simulink model "active_vehicle_ESP_Control"  (R2020a)
settings: Solver=ode4  StartTime=0.0  StopTime=inf  FixedStep=1e-3  RelTol=1e-3
InitFcn:
  | clear mex
model workspace (MAT data in the model file):
  inChnlList{1} = 'Driver_Demands.str_swa'
  inChnlList{2} = 'Subsystem_Activation.Internal_Steering_Column_Activity'
  inChnlList{3} = 'Driver_Demands.rack_displacement'
  inChnlList{4} = 'Driver_Demands.throttle'
  inChnlList{5} = 'Driver_Demands.gear'
  inChnlList{6} = 'Driver_Demands.clutch'
  inChnlList{7} = 'Driver_Demands.brake'
  inChnlList{8} = 'Driver_Demands.target_speed'
  inChnlList{9} = 'Driver_Demands.target_acc'
  inChnlList{10} = 'Brake_System_General.brk_mast_cyl_pres'
  inChnlList{11} = 'Brake_System_General.brk_bias_front'
  inChnlList{12} = 'ABS.Internal_ABS_Activity'
  inChnlList{13} = 'ABS.ABS_threshold'
  inChnlList{14} = 'Driver_Demands.user_maneuver_ID'
  inChnlList{15} = 'Driver_Demands.user_input_steering'
  inChnlList{16} = 'Driver_Demands.user_input_throttle'
  inChnlList{17} = 'Driver_Demands.user_input_braking'
  inChnlList{18} = 'Driver_Demands.user_input_gear'
  inChnlList{19} = 'Driver_Demands.user_input_clutch'
  inChnlList{20} = 'TCS.Internal_TCS_Activity'
  inChnlList{21} = 'TCS.TCS_threshold'
  inChnlList{22} = 'Friction.tire_mu.L1'
  inChnlList{23} = 'Friction.tire_mu.L2'
  inChnlList{24} = 'Friction.tire_mu.R1'
  inChnlList{25} = 'Friction.tire_mu.R2'
  inChnlList{26} = 'Subsystem_Activation.Internal_Brake_System_Activity.L1'
  inChnlList{27} = 'Brake_System.brk_mmag_sign.L1'
  inChnlList{28} = 'Brake_System.brk_mmag_unsign.L1'
  inChnlList{29} = 'Brake_System.brk_pres.L1'
  inChnlList{30} = 'Brake_System.brk_pres_gain.L1'
  inChnlList{31} = 'Brake_System.brk_mu.L1'
  inChnlList{32} = 'Subsystem_Activation.Internal_Brake_System_Activity.L2'
  inChnlList{33} = 'Brake_System.brk_mmag_sign.L2'
  inChnlList{34} = 'Brake_System.brk_mmag_unsign.L2'
  inChnlList{35} = 'Brake_System.brk_pres.L2'
  inChnlList{36} = 'Brake_System.brk_pres_gain.L2'
  inChnlList{37} = 'Brake_System.brk_mu.L2'
  inChnlList{38} = 'Subsystem_Activation.Internal_Brake_System_Activity.R1'
  inChnlList{39} = 'Brake_System.brk_mmag_sign.R1'
  inChnlList{40} = 'Brake_System.brk_mmag_unsign.R1'
  inChnlList{41} = 'Brake_System.brk_pres.R1'
  inChnlList{42} = 'Brake_System.brk_pres_gain.R1'
  inChnlList{43} = 'Brake_System.brk_mu.R1'
  inChnlList{44} = 'Subsystem_Activation.Internal_Brake_System_Activity.R2'
  inChnlList{45} = 'Brake_System.brk_mmag_sign.R2'
  inChnlList{46} = 'Brake_System.brk_mmag_unsign.R2'
  inChnlList{47} = 'Brake_System.brk_pres.R2'
  inChnlList{48} = 'Brake_System.brk_pres_gain.R2'
  inChnlList{49} = 'Brake_System.brk_mu.R2'
  inChnlList{50} = 'Hook.Fx.rear'
  inChnlList{51} = 'Hook.Fy.rear'
  inChnlList{52} = 'Hook.Fz.rear'
  inChnlList{53} = 'Hook.Mx.rear'
  inChnlList{54} = 'Hook.My.rear'
  inChnlList{55} = 'Hook.Mz.rear'
  inChnlList{56} = 'Rear_Steering_Actuator_disp.str_swa.left'
  inChnlList{57} = 'Rear_Steering_Actuator_disp.str_swa.right'
  inChnlList{58} = 'Steering.steer_at_spindle.L1'
  inChnlList{59} = 'Steering.steer_at_spindle.L2'
  inChnlList{60} = 'Steering.steer_at_spindle.R1'
  inChnlList{61} = 'Steering.steer_at_spindle.R2'
  inChnlList{62} = 'Subsystem_Activation.Internal_Clutch_Activity'
  inChnlList{63} = 'Subsystem_Activation.Internal_Engine_Activity'
  inChnlList{64} = 'Subsystem_Activation.Internal_Motor_to_Clutch_Activity'
  inChnlList{65} = 'Subsystem_Activation.Internal_Motor_to_GearBox_Activity'
  inChnlList{66} = 'Subsystem_Activation.Internal_Motor_to_CentralDifferential_Activity'
  inChnlList{67} = 'Subsystem_Activation.Internal_Motor_to_FrontDifferential_Activity'
  inChnlList{68} = 'Subsystem_Activation.Internal_Motor_to_RearDifferential_Activity'
  inChnlList{69} = 'Subsystem_Activation.Internal_Motor_to_FrontRightWheel_Activity'
  inChnlList{70} = 'Subsystem_Activation.Internal_Motor_to_FrontLeftWheel_Activity'
  inChnlList{71} = 'Subsystem_Activation.Internal_Motor_to_RearRightWheel_Activity'
  inChnlList{72} = 'Subsystem_Activation.Internal_Motor_to_RearLeftWheel_Activity'
  inChnlList{73} = 'Subsystem_Activation.Internal_Engine_Idle_MaxRev_Controls_Activity'
  inChnlList{74} = 'Subsystem_Activation.Internal_Gearbox_Activity'
  inChnlList{75} = 'Subsystem_Activation.Internal_CentralDifferential_Activity'
  inChnlList{76} = 'Subsystem_Activation.Internal_FrontDifferential_Activity'
  inChnlList{77} = 'Subsystem_Activation.Internal_RearDifferential_Activity'
  inChnlList{78} = 'Engine.engine_omega'
  inChnlList{79} = 'Engine.engine_max_trq'
  inChnlList{80} = 'Engine.engine_min_trq'
  inChnlList{81} = 'Engine.engine_trq'
  inChnlList{82} = 'Engine.clutch_inputplate_torque'
  inChnlList{83} = 'Engine.non_termic_engine_trq'
  inChnlList{84} = 'Engine.efficiency'
  inChnlList{85} = 'Engine.throttle_scaling'
  inChnlList{86} = 'Engine.control_mode'
  inChnlList{87} = 'Engine.throttle_offset'
  inChnlList{88} = 'GearBox.efficiency'
  inChnlList{89} = 'GearBox.transmission_ratio'
  inChnlList{90} = 'GearBox.diff_central_inputshaft_torque'
  inChnlList{91} = 'GearBox.clutch_outputplate_angle'
  inChnlList{92} = 'GearBox.clutch_outputplate_omega'
  inChnlList{93} = 'GearBox.clutch_outputplate_alpha'
  inChnlList{94} = 'GearBox.automatic_gearbox_shifting_mode'
  inChnlList{95} = 'Clutch.clutch_trq'
  inChnlList{96} = 'Clutch.gearbox_inputshaft_torque'
  inChnlList{97} = 'Clutch.inputplate_angle'
  inChnlList{98} = 'Clutch.inputplate_omega'
  inChnlList{99} = 'Clutch.inputplate_alpha'
  inChnlList{100} = 'Clutch.efficiency'
  inChnlList{101} = 'Differential_Central.efficiency'
  inChnlList{102} = 'Differential_Central.diff_front_inputshaft_torque'
  inChnlList{103} = 'Differential_Central.diff_rear_inputshaft_torque'
  inChnlList{104} = 'Differential_Central.gearbox_outputshaft_angle'
  inChnlList{105} = 'Differential_Central.gearbox_outputshaft_omega'
  inChnlList{106} = 'Differential_Central.gearbox_outputshaft_alpha'
  inChnlList{107} = 'Differential_Front.efficiency'
  inChnlList{108} = 'Differential_Front.wheel_front_left_torque'
  inChnlList{109} = 'Differential_Front.wheel_front_right_torque'
  inChnlList{110} = 'Differential_Front.diff_central_front_outputshaft_angle'
  inChnlList{111} = 'Differential_Front.diff_central_front_outputshaft_omega'
  inChnlList{112} = 'Differential_Front.diff_central_front_outputshaft_alpha'
  inChnlList{113} = 'Differential_Rear.efficiency'
  inChnlList{114} = 'Differential_Rear.wheel_rear_left_torque'
  inChnlList{115} = 'Differential_Rear.wheel_rear_right_torque'
  inChnlList{116} = 'Differential_Rear.diff_central_rear_outputshaft_angle'
  inChnlList{117} = 'Differential_Rear.diff_central_rear_outputshaft_omega'
  inChnlList{118} = 'Differential_Rear.diff_central_rear_outputshaft_alpha'
  inChnlList{119} = 'Generic_Engine_to_Clutch.transmission_ratio'
  inChnlList{120} = 'Generic_Engine_to_Clutch.regeneration_factor'
  inChnlList{121} = 'Generic_Engine_to_Clutch.throttle_scaling'
  inChnlList{122} = 'Generic_Engine_to_Clutch.control_mode'
  inChnlList{123} = 'Generic_Engine_to_Clutch.throttle_offset'
  inChnlList{124} = 'Generic_Engine_to_Clutch.efficiency'
  inChnlList{125} = 'Generic_Engine_to_Clutch.engine_torque'
  inChnlList{126} = 'Generic_Engine_to_Clutch.engine_max_torque'
  inChnlList{127} = 'Generic_Engine_to_Clutch.engine_min_torque'
  inChnlList{128} = 'Generic_Engine_to_Gearbox.transmission_ratio'
  inChnlList{129} = 'Generic_Engine_to_Gearbox.regeneration_factor'
  inChnlList{130} = 'Generic_Engine_to_Gearbox.throttle_scaling'
  inChnlList{131} = 'Generic_Engine_to_Gearbox.control_mode'
  inChnlList{132} = 'Generic_Engine_to_Gearbox.throttle_offset'
  inChnlList{133} = 'Generic_Engine_to_Gearbox.efficiency'
  inChnlList{134} = 'Generic_Engine_to_Gearbox.engine_torque'
  inChnlList{135} = 'Generic_Engine_to_Gearbox.engine_max_torque'
  inChnlList{136} = 'Generic_Engine_to_Gearbox.engine_min_torque'
  inChnlList{137} = 'Generic_Engine_to_Central_Differential.transmission_ratio'
  inChnlList{138} = 'Generic_Engine_to_Central_Differential.reverse_mode'
  inChnlList{139} = 'Generic_Engine_to_Central_Differential.regeneration_factor'
  inChnlList{140} = 'Generic_Engine_to_Central_Differential.throttle_scaling'
  inChnlList{141} = 'Generic_Engine_to_Central_Differential.control_mode'
  inChnlList{142} = 'Generic_Engine_to_Central_Differential.throttle_offset'
  inChnlList{143} = 'Generic_Engine_to_Central_Differential.efficiency'
  inChnlList{144} = 'Generic_Engine_to_Central_Differential.engine_torque'
  inChnlList{145} = 'Generic_Engine_to_Central_Differential.engine_max_torque'
  inChnlList{146} = 'Generic_Engine_to_Central_Differential.engine_min_torque'
  inChnlList{147} = 'Generic_Engine_to_Front_Differential.transmission_ratio'
  inChnlList{148} = 'Generic_Engine_to_Front_Differential.reverse_mode'
  inChnlList{149} = 'Generic_Engine_to_Front_Differential.regeneration_factor'
  inChnlList{150} = 'Generic_Engine_to_Front_Differential.throttle_scaling'
  inChnlList{151} = 'Generic_Engine_to_Front_Differential.control_mode'
  inChnlList{152} = 'Generic_Engine_to_Front_Differential.throttle_offset'
  inChnlList{153} = 'Generic_Engine_to_Front_Differential.efficiency'
  inChnlList{154} = 'Generic_Engine_to_Front_Differential.engine_torque'
  inChnlList{155} = 'Generic_Engine_to_Front_Differential.engine_max_torque'
  inChnlList{156} = 'Generic_Engine_to_Front_Differential.engine_min_torque'
  inChnlList{157} = 'Generic_Engine_to_Rear_Differential.transmission_ratio'
  inChnlList{158} = 'Generic_Engine_to_Rear_Differential.reverse_mode'
  inChnlList{159} = 'Generic_Engine_to_Rear_Differential.regeneration_factor'
  inChnlList{160} = 'Generic_Engine_to_Rear_Differential.throttle_scaling'
  inChnlList{161} = 'Generic_Engine_to_Rear_Differential.control_mode'
  inChnlList{162} = 'Generic_Engine_to_Rear_Differential.throttle_offset'
  inChnlList{163} = 'Generic_Engine_to_Rear_Differential.efficiency'
  inChnlList{164} = 'Generic_Engine_to_Rear_Differential.engine_torque'
  inChnlList{165} = 'Generic_Engine_to_Rear_Differential.engine_max_torque'
  inChnlList{166} = 'Generic_Engine_to_Rear_Differential.engine_min_torque'
  inChnlList{167} = 'Generic_Engine_to_Front_Right_Wheel.transmission_ratio'
  inChnlList{168} = 'Generic_Engine_to_Front_Right_Wheel.reverse_mode'
  inChnlList{169} = 'Generic_Engine_to_Front_Right_Wheel.regeneration_factor'
  inChnlList{170} = 'Generic_Engine_to_Front_Right_Wheel.throttle_scaling'
  inChnlList{171} = 'Generic_Engine_to_Front_Right_Wheel.control_mode'
  inChnlList{172} = 'Generic_Engine_to_Front_Right_Wheel.throttle_offset'
  inChnlList{173} = 'Generic_Engine_to_Front_Right_Wheel.efficiency'
  inChnlList{174} = 'Generic_Engine_to_Front_Right_Wheel.engine_torque'
  inChnlList{175} = 'Generic_Engine_to_Front_Right_Wheel.engine_max_torque'
  inChnlList{176} = 'Generic_Engine_to_Front_Right_Wheel.engine_min_torque'
  inChnlList{177} = 'Generic_Engine_to_Front_Left_Wheel.transmission_ratio'
  inChnlList{178} = 'Generic_Engine_to_Front_Left_Wheel.reverse_mode'
  inChnlList{179} = 'Generic_Engine_to_Front_Left_Wheel.regeneration_factor'
  inChnlList{180} = 'Generic_Engine_to_Front_Left_Wheel.throttle_scaling'
  inChnlList{181} = 'Generic_Engine_to_Front_Left_Wheel.control_mode'
  inChnlList{182} = 'Generic_Engine_to_Front_Left_Wheel.throttle_offset'
  inChnlList{183} = 'Generic_Engine_to_Front_Left_Wheel.efficiency'
  inChnlList{184} = 'Generic_Engine_to_Front_Left_Wheel.engine_torque'
  inChnlList{185} = 'Generic_Engine_to_Front_Left_Wheel.engine_max_torque'
  inChnlList{186} = 'Generic_Engine_to_Front_Left_Wheel.engine_min_torque'
  inChnlList{187} = 'Generic_Engine_to_Rear_Right_Wheel.transmission_ratio'
  inChnlList{188} = 'Generic_Engine_to_Rear_Right_Wheel.reverse_mode'
  inChnlList{189} = 'Generic_Engine_to_Rear_Right_Wheel.regeneration_factor'
  inChnlList{190} = 'Generic_Engine_to_Rear_Right_Wheel.throttle_scaling'
  inChnlList{191} = 'Generic_Engine_to_Rear_Right_Wheel.control_mode'
  inChnlList{192} = 'Generic_Engine_to_Rear_Right_Wheel.throttle_offset'
  inChnlList{193} = 'Generic_Engine_to_Rear_Right_Wheel.efficiency'
  inChnlList{194} = 'Generic_Engine_to_Rear_Right_Wheel.engine_torque'
  inChnlList{195} = 'Generic_Engine_to_Rear_Right_Wheel.engine_max_torque'
  inChnlList{196} = 'Generic_Engine_to_Rear_Right_Wheel.engine_min_torque'
  inChnlList{197} = 'Generic_Engine_to_Rear_Left_Wheel.transmission_ratio'
  inChnlList{198} = 'Generic_Engine_to_Rear_Left_Wheel.reverse_mode'
  inChnlList{199} = 'Generic_Engine_to_Rear_Left_Wheel.regeneration_factor'
  inChnlList{200} = 'Generic_Engine_to_Rear_Left_Wheel.throttle_scaling'
  inChnlList{201} = 'Generic_Engine_to_Rear_Left_Wheel.control_mode'
  inChnlList{202} = 'Generic_Engine_to_Rear_Left_Wheel.throttle_offset'
  inChnlList{203} = 'Generic_Engine_to_Rear_Left_Wheel.efficiency'
  inChnlList{204} = 'Generic_Engine_to_Rear_Left_Wheel.engine_torque'
  inChnlList{205} = 'Generic_Engine_to_Rear_Left_Wheel.engine_max_torque'
  inChnlList{206} = 'Generic_Engine_to_Rear_Left_Wheel.engine_min_torque'
  inChnlList{207} = 'Antiroll_Bar.activity_flag.front'
  inChnlList{208} = 'Antiroll_Bar.activity_flag.rear'
  inChnlList{209} = 'Antiroll_Bar.force.front'
  inChnlList{210} = 'Antiroll_Bar.force.rear'
  inChnlList{211} = 'Subsystem_Activation.Internal_Aero_Activity'
  inChnlList{212} = 'Aerodynamic.my_scaling'
  inChnlList{213} = 'Aerodynamic.fx_central_scaling'
  inChnlList{214} = 'Aerodynamic.fz_front_scaling'
  inChnlList{215} = 'Aerodynamic.fz_rear_scaling'
  inChnlList{216} = 'Aerodynamic.fx_front'
  inChnlList{217} = 'Aerodynamic.fy_front'
  inChnlList{218} = 'Aerodynamic.fz_front'
  inChnlList{219} = 'Aerodynamic.fx_rear'
  inChnlList{220} = 'Aerodynamic.fy_rear'
  inChnlList{221} = 'Aerodynamic.fz_rear'
  inChnlList{222} = 'Aerodynamic.fx_center'
  inChnlList{223} = 'Aerodynamic.fy_center'
  inChnlList{224} = 'Aerodynamic.fz_center'
  inChnlList{225} = 'Aerodynamic.mx'
  inChnlList{226} = 'Aerodynamic.my'
  inChnlList{227} = 'Aerodynamic.mz'
  inChnlList{228} = 'Irregularity.road.L1'
  inChnlList{229} = 'Irregularity.road.L2'
  inChnlList{230} = 'Irregularity.road.R1'
  inChnlList{231} = 'Irregularity.road.R2'
  inChnlList{232} = 'Main_Damper.force.L1'
  inChnlList{233} = 'Main_Damper.activity_flag.L1'
  inChnlList{234} = 'Main_Damper.force.L2'
  inChnlList{235} = 'Main_Damper.activity_flag.L2'
  inChnlList{236} = 'Main_Damper.force.R1'
  inChnlList{237} = 'Main_Damper.activity_flag.R1'
  inChnlList{238} = 'Main_Damper.force.R2'
  inChnlList{239} = 'Main_Damper.activity_flag.R2'
  inChnlList{240} = 'Main_Spring.force.L1'
  inChnlList{241} = 'Main_Spring.activity_flag.L1'
  inChnlList{242} = 'Main_Spring.force.L2'
  inChnlList{243} = 'Main_Spring.activity_flag.L2'
  inChnlList{244} = 'Main_Spring.force.R1'
  inChnlList{245} = 'Main_Spring.activity_flag.R1'
  inChnlList{246} = 'Main_Spring.force.R2'
  inChnlList{247} = 'Main_Spring.activity_flag.R2'
  inChnlList{248} = 'Main_Bumpstop.force.L1'
  inChnlList{249} = 'Main_Bumpstop.activity_flag.L1'
  inChnlList{250} = 'Main_Bumpstop.force.L2'
  inChnlList{251} = 'Main_Bumpstop.activity_flag.L2'
  inChnlList{252} = 'Main_Bumpstop.force.R1'
  inChnlList{253} = 'Main_Bumpstop.activity_flag.R1'
  inChnlList{254} = 'Main_Bumpstop.force.R2'
  inChnlList{255} = 'Main_Bumpstop.activity_flag.R2'
  inChnlList{256} = 'Main_Reboundstop.force.L1'
  inChnlList{257} = 'Main_Reboundstop.activity_flag.L1'
  inChnlList{258} = 'Main_Reboundstop.force.L2'
  inChnlList{259} = 'Main_Reboundstop.activity_flag.L2'
  inChnlList{260} = 'Main_Reboundstop.force.R1'
  inChnlList{261} = 'Main_Reboundstop.activity_flag.R1'
  inChnlList{262} = 'Main_Reboundstop.force.R2'
  inChnlList{263} = 'Main_Reboundstop.activity_flag.R2'
  inChnlList{264} = 'Auxiliary_vertical.force.L1'
  inChnlList{265} = 'Auxiliary_vertical.activity_flag.L1'
  inChnlList{266} = 'Auxiliary_vertical.force.L2'
  inChnlList{267} = 'Auxiliary_vertical.activity_flag.L2'
  inChnlList{268} = 'Auxiliary_vertical.force.R1'
  inChnlList{269} = 'Auxiliary_vertical.activity_flag.R1'
  inChnlList{270} = 'Auxiliary_vertical.force.R2'
  inChnlList{271} = 'Auxiliary_vertical.activity_flag.R2'
  inChnlList{272} = 'Main_Inerter.force.L1'
  inChnlList{273} = 'Main_Inerter.activity_flag.L1'
  inChnlList{274} = 'Main_Inerter.force.L2'
  inChnlList{275} = 'Main_Inerter.activity_flag.L2'
  inChnlList{276} = 'Main_Inerter.force.R1'
  inChnlList{277} = 'Main_Inerter.activity_flag.R1'
  inChnlList{278} = 'Main_Inerter.force.R2'
  inChnlList{279} = 'Main_Inerter.activity_flag.R2'
  inChnlList{280} = 'Third_Element.Damper_force.front'
  inChnlList{281} = 'Third_Element.Damper_activity_flag.front'
  inChnlList{282} = 'Third_Element.Damper_force.rear'
  inChnlList{283} = 'Third_Element.Damper_activity_flag.rear'
  inChnlList{284} = 'Third_Element.Spring.front'
  inChnlList{285} = 'Third_Element.Spring_activity_flag.front'
  inChnlList{286} = 'Third_Element.Spring.rear'
  inChnlList{287} = 'Third_Element.Spring_activity_flag.rear'
  inChnlList{288} = 'Mono_Element.Damper.front'
  inChnlList{289} = 'Mono_Element.Damper_activity_flag.front'
  inChnlList{290} = 'Mono_Element.Damper.rear'
  inChnlList{291} = 'Mono_Element.Damper_activity_flag.rear'
  inChnlList{292} = 'Mono_Element.Inerter.front'
  inChnlList{293} = 'Mono_Element.Inerter_activity_flag.front'
  inChnlList{294} = 'Mono_Element.Inerter.rear'
  inChnlList{295} = 'Mono_Element.Inerter_activity_flag.rear'
  inChnlList{296} = 'Mono_Element.Spring.front'
  inChnlList{297} = 'Mono_Element.Spring_activity_flag.front'
  inChnlList{298} = 'Mono_Element.Spring.rear'
  inChnlList{299} = 'Mono_Element.Spring_activity_flag.rear'
  inChnlList{300} = 'Mono_Element.Bumpstop_Spring.front'
  inChnlList{301} = 'Mono_Element.Bumpstop_Spring_activity_flag.front'
  inChnlList{302} = 'Mono_Element.Bumpstop_Spring.rear'
  inChnlList{303} = 'Mono_Element.Bumpstop_Spring_activity_flag.rear'
  inChnlList{304} = 'Mono_Element.Reboundstop_Spring.front'
  inChnlList{305} = 'Mono_Element.Reboundstop_Spring_activity_flag.front'
  inChnlList{306} = 'Mono_Element.Reboundstop_Spring.rear'
  inChnlList{307} = 'Mono_Element.Reboundstop_Spring_activity_flag.rear'
  inChnlList{308} = 'Mono_Element.Bumpstop_Damper.front'
  inChnlList{309} = 'Mono_Element.Bumpstop_Damper_activity_flag.front'
  inChnlList{310} = 'Mono_Element.Bumpstop_Damper.rear'
  inChnlList{311} = 'Mono_Element.Bumpstop_Damper_activity_flag.rear'
  inChnlList{312} = 'Mono_Element.Reboundstop_Damper.front'
  inChnlList{313} = 'Mono_Element.Reboundstop_Damper_activity_flag.front'
  inChnlList{314} = 'Mono_Element.Reboundstop_Damper.rear'
  inChnlList{315} = 'Mono_Element.Reboundstop_Damper_activity_flag.rear'
  inChnlList{316} = 'Mono_Element.Roll_Damper.front'
  inChnlList{317} = 'Mono_Element.Roll_Damper_activity_flag.front'
  inChnlList{318} = 'Mono_Element.Roll_Damper.rear'
  inChnlList{319} = 'Mono_Element.Roll_Damper_activity_flag.rear'
  inChnlList{320} = 'Subsystem_Activation.Tire_Force_x.L1'
  inChnlList{321} = 'Subsystem_Activation.Tire_Force_y.L1'
  inChnlList{322} = 'Subsystem_Activation.Tire_Force_z.L1'
  inChnlList{323} = 'Subsystem_Activation.Tire_Moment_x.L1'
  inChnlList{324} = 'Subsystem_Activation.Tire_Moment_y.L1'
  inChnlList{325} = 'Subsystem_Activation.Tire_Moment_z.L1'
  inChnlList{326} = 'Tire_Force.Fx.L1'
  inChnlList{327} = 'Tire_Force.Fy.L1'
  inChnlList{328} = 'Tire_Force.Fz.L1'
  inChnlList{329} = 'Tire_Moment.Mx.L1'
  inChnlList{330} = 'Tire_Moment.My.L1'
  inChnlList{331} = 'Tire_Moment.Mz.L1'
  inChnlList{332} = 'Subsystem_Activation.Tire_Force_x.L2'
  inChnlList{333} = 'Subsystem_Activation.Tire_Force_y.L2'
  inChnlList{334} = 'Subsystem_Activation.Tire_Force_z.L2'
  inChnlList{335} = 'Subsystem_Activation.Tire_Moment_x.L2'
  inChnlList{336} = 'Subsystem_Activation.Tire_Moment_y.L2'
  inChnlList{337} = 'Subsystem_Activation.Tire_Moment_z.L2'
  inChnlList{338} = 'Tire_Force.Fx.L2'
  inChnlList{339} = 'Tire_Force.Fy.L2'
  inChnlList{340} = 'Tire_Force.Fz.L2'
  inChnlList{341} = 'Tire_Moment.Mx.L2'
  inChnlList{342} = 'Tire_Moment.My.L2'
  inChnlList{343} = 'Tire_Moment.Mz.L2'
  inChnlList{344} = 'Subsystem_Activation.Tire_Force_x.R1'
  inChnlList{345} = 'Subsystem_Activation.Tire_Force_y.R1'
  inChnlList{346} = 'Subsystem_Activation.Tire_Force_z.R1'
  inChnlList{347} = 'Subsystem_Activation.Tire_Moment_x.R1'
  inChnlList{348} = 'Subsystem_Activation.Tire_Moment_y.R1'
  inChnlList{349} = 'Subsystem_Activation.Tire_Moment_z.R1'
  inChnlList{350} = 'Tire_Force.Fx.R1'
  inChnlList{351} = 'Tire_Force.Fy.R1'
  inChnlList{352} = 'Tire_Force.Fz.R1'
  inChnlList{353} = 'Tire_Moment.Mx.R1'
  inChnlList{354} = 'Tire_Moment.My.R1'
  inChnlList{355} = 'Tire_Moment.Mz.R1'
  inChnlList{356} = 'Subsystem_Activation.Tire_Force_x.R2'
  inChnlList{357} = 'Subsystem_Activation.Tire_Force_y.R2'
  inChnlList{358} = 'Subsystem_Activation.Tire_Force_z.R2'
  inChnlList{359} = 'Subsystem_Activation.Tire_Moment_x.R2'
  inChnlList{360} = 'Subsystem_Activation.Tire_Moment_y.R2'
  inChnlList{361} = 'Subsystem_Activation.Tire_Moment_z.R2'
  inChnlList{362} = 'Tire_Force.Fx.R2'
  inChnlList{363} = 'Tire_Force.Fy.R2'
  inChnlList{364} = 'Tire_Force.Fz.R2'
  inChnlList{365} = 'Tire_Moment.Mx.R2'
  inChnlList{366} = 'Tire_Moment.My.R2'
  inChnlList{367} = 'Tire_Moment.Mz.R2'
  inChnlList{368} = 'Wheel_driving.moment.L1'
  inChnlList{369} = 'Wheel_driving.moment.L2'
  inChnlList{370} = 'Wheel_driving.moment.R1'
  inChnlList{371} = 'Wheel_driving.moment.R2'
  inChnlList{372} = 'Ext_Body.force.X'
  inChnlList{373} = 'Ext_Body.force.Y'
  inChnlList{374} = 'Ext_Body.force.Z'
  inChnlList{375} = 'Ext_Body.moment.X'
  inChnlList{376} = 'Ext_Body.moment.Y'
  inChnlList{377} = 'Ext_Body.moment.Z'
  inChnlList{378} = 'Ext_Ground.force.X'
  inChnlList{379} = 'Ext_Ground.force.Y'
  inChnlList{380} = 'Ext_Ground.force.Z'
  inChnlList{381} = 'Ext_Ground.moment.X'
  inChnlList{382} = 'Ext_Ground.moment.Y'
  inChnlList{383} = 'Ext_Ground.moment.Z'
  inChnlList{384} = 'Ext_Tracking.force.X'
  inChnlList{385} = 'Ext_Tracking.force.Y'
  inChnlList{386} = 'Ext_Tracking.moment.X'
  inChnlList{387} = 'Ext_Tracking.moment.Y'
  inChnlList{388} = 'steer_assist.force'
  inChnlList{389} = 'steer_assist.torque'
  inChnlList{390} = 'steering_torque.torque'
  inChnlList{391} = 'steering_assist.motor_torque'
  inChnlList{392} = 'Steering_System.auxiliary_steering_torque'
  inChnlListInternal : object (value not decoded)
  outChnlList : object (value not decoded)
  outChnlListInternal : object (value not decoded)
undefined symbols (not defined in the file or in its folder): DiscIntNeverNeededParam, vicrt_initcallback, vicrt_initmexcallback, vicrt_inputfile, vicrt_simulationmanager
libraries: simulink x1
(part 1 of 6)
settings Model: Creator=mcava  LastModifiedBy=lucas
settings DataIOCC: LimitDataPoints=on  SaveFormat=Array  SignalLoggingSaveFormat=ModelDataLogs  ReturnWorkspaceOutputs=off  SignalLoggingName=sigsOut
settings OptimizationCC: ExpressionDepthLimit=2147483647  InitFltsAndDblsToZero=on  LifeSpan=inf
settings DebuggingCC: SignalInfNanChecking=warning  SaveWithParameterizedLinksMsg=none  UnderspecifiedInitializationDetection=Classic  MergeDetectMultiDrivingBlocksExec=none  SignalResolutionControl=TryResolveAllWithWarning  MultiTaskDSMMsg=warning  MultiTaskCondExecSysMsg=none  FcnCallInpInsideContextMsg=warning  AllowSymbolicDim=off  StateNameClashWarn=warning  SFUnexpectedBacktrackingDiag=warning  SFNoUnconditionalDefaultTransitionDiag=warning  SFExecutionAtInitializationDiag=none  ArithmeticOperatorsInVariantConditions=warning
settings HardwareCC: ProdBitPerPointer=32  ProdBitPerSizeT=32  ProdBitPerPtrDiffT=32  ProdLargestAtomicFloat=None  ProdIntDivRoundTo=Undefined  ProdEndianess=Unspecified  ProdWordSize=32  ProdHWDeviceType=32-bit Generic  TargetBitPerPointer=64  TargetBitPerSizeT=64  TargetBitPerPtrDiffT=64  TargetLongLongMode=on  TargetIntDivRoundTo=Zero  TargetEndianess=LittleEndian  TargetWordSize=64  TargetHWDeviceType=MATLAB Host  ProdEqTarget=off
settings ModelReferenceCC: PropagateSignalLabelsOutOfModel=off
settings SFSimCC: SimUseLocalCustomCode=off  SimParseCustomCode=off  CustomCodeUndefinedFunction=UseInterfaceOnly
settings RTWCC: Description=VI-CarRealTime Solver Plugin V1.0  SystemTargetFile=vicrt_plugin.tlc  TemplateMakefile=vicrt_plugin_vcx64.tmf  PostCodeGenCommand=if strcmp(get_param(bdroot,'TemplateMakefile'),'vicrt_plugin_ccur.tmf'),copyfile([matlabroot,filesep,'rtw',filesep,'c',filesep,'tools',filesep,'unixtools.mk'],'unixtools.mk'),end  RTWVerbose=off  RTWUseLocalCustomCode=off
settings CodeAppCC: GenerateComments=off  MaxIdLength=80  SimulinkBlockComments=off
settings STFCustomTargetCC: ModelReferenceCompliant=off  CombineOutputUpdateFcns=on  MatFileLogging=on  SystemTargetFile=vicrt_plugin.tlc
settings GRTTargetCC: TargetLangStandard=C89/C90 (ANSI)  ModelReferenceCompliant=off  ParMdlRefBuildCompliant=off  CompOptLevelCompliant=off  ConcurrentExecutionCompliant=off  CPPClassGenCompliant=off  UseToolchainInfoCompliant=off  RTWCAPIParams=on
settings ConfigComp: CovMetricSettings=dw  CovHtmlReporting=on  CovSaveCumulativeToWorkspaceVar=on  CovSaveSingleToWorkspaceVar=on  CovExternalEMLEnable=off

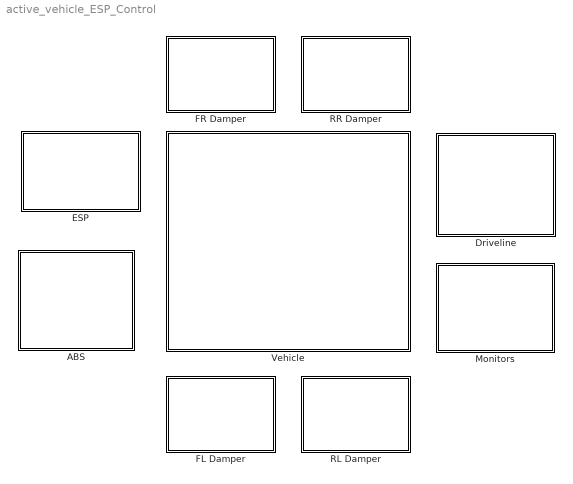
== system active_vehicle_ESP_Control ==
  ABS : Subsystem  mask{ABSActive=on}
      mask prompts: ABSActive "Active"
      mask Display: image(imread('abs.jpg'))
  Driveline : Subsystem
      mask Display: image(imread('driveline.jpg'))
  ESP : Subsystem  mask(ESP Controller){ESPActive=off, WheelBase=2.838, SteeringRatio=(7.85/54)}
      mask prompts: ESPActive "Active"
      mask help:
      | Active toggle switches ESP On/Off
      | WheelBase and SteeringRatio parameters are used  to calculate theorical Vehicle Yaw Rate.
      mask Display: image(imread('esp.jpg'))
  FL Damper : Subsystem  mask{FLDamperActive=off}
      mask prompts: FLDamperActive "Active"
      mask Display: image(imread('damper.jpg'))
  FR Damper : Subsystem  mask{FRDamperActive=off}
      mask prompts: FRDamperActive "Active"
      mask Display: image(imread('damper.jpg'))
  Monitors : Subsystem
      mask Display: image(imread('monitors.jpg'))
  RL Damper : Subsystem  mask{RLDamperActive=off}
      mask prompts: RLDamperActive "Active"
      mask Display: image(imread('damper.jpg'))
  RR Damper : Subsystem  mask{RRDamperActive=off}
      mask prompts: RRDamperActive "Active"
      mask Display: image(imread('damper.jpg'))
  Vehicle : Subsystem
      mask Display: image(imread('vehicle.jpg'))

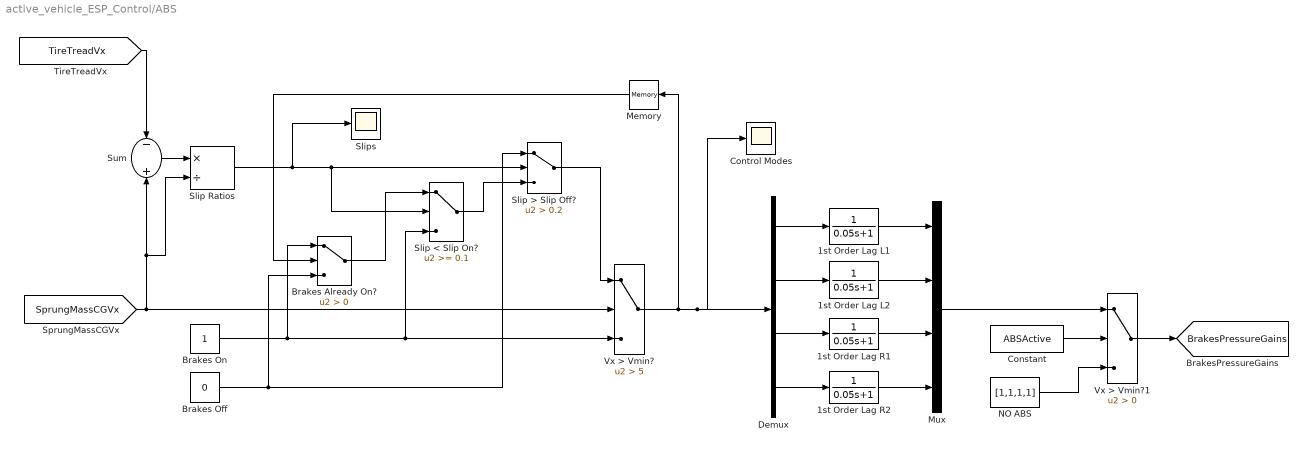
== system active_vehicle_ESP_Control/ABS ==
  1st Order Lag L1 : TransferFcn  Denominator="[0.05  1]"
  1st Order Lag L2 : TransferFcn  Denominator="[0.05  1]"
  1st Order Lag R1 : TransferFcn  Denominator="[0.05  1]"
  1st Order Lag R2 : TransferFcn  Denominator="[0.05  1]"
  Brakes Already On? : Switch  Criteria=u2 > Threshold  SaturateOnIntegerOverflow=on
  Brakes Off : Constant  Value=0
  Brakes On : Constant
  Constant : Constant  Value=ABSActive
  Control Modes : Scope
  Demux : Demux
      settings: DisplayOption=none
  Memory : Memory  InitialCondition=[1,1,1,1]
  Mux : Mux
  NO ABS : Constant  Value=[1,1,1,1]
  Slip < Slip On? : Switch  Threshold=0.1  SaturateOnIntegerOverflow=on
  Slip > Slip Off? : Switch  Criteria=u2 > Threshold  Threshold=0.2  SaturateOnIntegerOverflow=on
  Slip Ratios : Product  Inputs=*/  SaturateOnIntegerOverflow=on  OutDataTypeStr=Inherit: Same as first input
  Slips : Scope
  Sum : Sum  Inputs=-+  SaturateOnIntegerOverflow=on  OutDataTypeStr=Inherit: Same as first input
  Vx > Vmin? : Switch  Criteria=u2 > Threshold  Threshold=5  SaturateOnIntegerOverflow=on
  Vx > Vmin?1 : Switch  Criteria=u2 > Threshold  SaturateOnIntegerOverflow=on
  tag scope: BrakesPressureGains=global
  wires:
  Sum/1 -> Slip Ratios/1
  [SprungMassCGVx] -> Slip Ratios/2, Sum/2, Vx > Vmin?/2
  Vx > Vmin?/1 -> Memory/1, Control Modes/1, Demux/1
  Slip > Slip Off?/1 -> Vx > Vmin?/1
  Brakes On/1 -> Brakes Already On?/1, Vx > Vmin?/3, Slip < Slip On?/3
  Brakes Off/1 -> Slip > Slip Off?/1, Brakes Already On?/3
  Slip Ratios/1 -> Slips/1, Slip > Slip Off?/2, Slip < Slip On?/2
  Slip < Slip On?/1 -> Slip > Slip Off?/3
  Memory/1 -> Brakes Already On?/2
  Brakes Already On?/1 -> Slip < Slip On?/1
  Demux/4 -> 1st Order Lag R2/1
  Demux/3 -> 1st Order Lag R1/1
  Demux/2 -> 1st Order Lag L2/1
  Demux/1 -> 1st Order Lag L1/1
  1st Order Lag L1/1 -> Mux/1
  1st Order Lag L2/1 -> Mux/2
  1st Order Lag R1/1 -> Mux/3
  1st Order Lag R2/1 -> Mux/4
  Mux/1 -> Vx > Vmin?1/1
  [TireTreadVx] -> Sum/1
  Constant/1 -> Vx > Vmin?1/2
  Vx > Vmin?1/1 -> [BrakesPressureGains]
  NO ABS/1 -> Vx > Vmin?1/3

== system active_vehicle_ESP_Control/Driveline ==
  Clutch : Subsystem  mask{UserClutchActive=off}
      mask prompts: UserClutchActive "Active"
      mask Display: image(imread('clutch.jpg'))
  Engine : Subsystem  mask{UserEngineActive=off}
      mask prompts: UserEngineActive "Active"
      mask Display: image(imread('engine.jpg'))
  GearBox : Subsystem  mask{UserGearBoxActive=off}
      mask prompts: UserGearBoxActive "Active"
      mask Display: image(imread('gearbox.jpg'))
  Rear Differential : Subsystem  mask{RearDifferentialActive=off, DriveRatio=3.7}
      mask prompts: RearDifferentialActive "Active"; DriveRatio "Drive Ratio"
      mask Display: image(imread('differential.jpg'))

== system active_vehicle_ESP_Control/ESP ==
  Constant : Constant  Value=ESPActive
  ESP : Subsystem  TreatAsAtomicUnit=on
  Memory : Memory  InitialCondition=[0,0,0,0]
  Mux : Mux
  Product : Product  RndMeth=Zero  OutDataTypeStr=Inherit: Same as first input
  tag scope: ESPUnsignedTorques=global, ThrottleOff=global
  wires:
  ESP/5(ThrottleOff) -> [ThrottleOff]
  Memory/1 -> [ESPUnsignedTorques]
  ESP/3(RF) -> Mux/3
  ESP/2(LR) -> Mux/2
  Product/1 -> Memory/1
  Constant/1 -> Product/1
  Mux/1 -> Product/2
  ESP/1(LF) -> Mux/1
  ESP/4(RR) -> Mux/4
  [SideSlipAngle] -> ESP/1(SIde_slip)
  [YawRate] -> ESP/2("yawr ")
  [SteeringDemand] -> ESP/3(steer)
  [LongitudinalVelocity] -> ESP/4(Vx)

== system active_vehicle_ESP_Control/FL Damper ==
  "C " : Gain  Gain=4000  OutDataTypeStr=Inherit: Same as input  ParamDataTypeStr=Inherit: Same as input
  Constant : Constant  Value=FLDamperActive
  Data Type Conversion : DataTypeConversion
  DmpF Lookup : Lookup  InputValues=|  Table=|
      InputValues=|
      | [ -1.5800000e+000 -1.0200000e+000 -7.7000000e-001 -5.1000000e-001 -3.8000000e-001 -2.5000000e-001 -1.3000000e-001 -5.0000000e-002 -3.0000000e-002 -1.0000000e-002  0.0000000e+000  1.0000000e-002  3.0000000e-002  5.0000000e-002  1.3000000e-001  2.6000000e-001  3.8000000e-001  5.1000000e-001  7.8000000e-001  1.0400000e+000  1.6200000e+000	
      | ]
      Table=|
      | [ -3.2605700e+003 -2.6592520e+003 -2.3311553e+003 -1.9825529e+003 -1.7569865e+003 -1.5314201e+003 -1.2853477e+003 -8.9573310e+002 -7.0015000e+002 -3.9192000e+002  0.0000000e+000  1.7058070e+002  4.3715920e+002  6.6272540e+002  1.0113279e+003  1.4419546e+003  1.6470150e+003  1.7905570e+003  2.1107987e+003  2.4057380e+003  3.1155941e+003	
      | ]
  Gain : Gain  Gain=1.2  OutDataTypeStr=Inherit: Same as input  ParamDataTypeStr=Inherit: Same as input
  Lin/Spline switch : ManualSwitch
  Logical Operator : Logic  Operator=NOT  AllPortsSameDT=off  OutDataTypeStr=boolean
  Memory : Memory
  Minus1 : UnaryMinus
  Minus2 : UnaryMinus
  Product : Product  RndMeth=Zero  OutDataTypeStr=Inherit: Same as first input
  Product1 : Product  RndMeth=Zero  OutDataTypeStr=Inherit: Same as first input
  Vx Lookup : Lookup  InputValues=|  Table=|
      InputValues=|
      | [ -5e-2 -1e-2 -5e-3 0 5e-3 1e-2 5e-2
      | ]
      Table=|
      | [ 1 1 1 0.2 1 1 1
      | ]
  tag scope: FLDamperForce=global, InternalFLDamperActive=global
  wires:
  Product/1 -> [FLDamperForce]
  Memory/1 -> Product/1
  Lin/Spline switch/1 -> Memory/1
  [FLDamperVelocity] -> Minus2/1, "C "/1
  Minus2/1 -> DmpF Lookup/1
  DmpF Lookup/1 -> Minus1/1
  "C "/1 -> Lin/Spline switch/2
  Minus1/1 -> Product1/2
  Product1/1 -> Lin/Spline switch/1
  Vx Lookup/1 -> Gain/1
  Gain/1 -> Product1/1
  [VerticalVelocity] -> Vx Lookup/1
  Data Type Conversion/1 -> [InternalFLDamperActive]
  Constant/1 -> Product/2, Logical Operator/1
  Logical Operator/1 -> Data Type Conversion/1

== system active_vehicle_ESP_Control/FR Damper ==
  "C " : Gain  Gain=4000  OutDataTypeStr=Inherit: Same as input  ParamDataTypeStr=Inherit: Same as input
  Constant : Constant  Value=FRDamperActive
  Data Type Conversion : DataTypeConversion
  DmpF Lookup : Lookup  InputValues=|  Table=|
      InputValues=|
      | [ -1.5800000e+000 -1.0200000e+000 -7.7000000e-001 -5.1000000e-001 -3.8000000e-001 -2.5000000e-001 -1.3000000e-001 -5.0000000e-002 -3.0000000e-002 -1.0000000e-002  0.0000000e+000  1.0000000e-002  3.0000000e-002  5.0000000e-002  1.3000000e-001  2.6000000e-001  3.8000000e-001  5.1000000e-001  7.8000000e-001  1.0400000e+000  1.6200000e+000	
      | ]
      Table=|
      | [ -3.2605700e+003 -2.6592520e+003 -2.3311553e+003 -1.9825529e+003 -1.7569865e+003 -1.5314201e+003 -1.2853477e+003 -8.9573310e+002 -7.0015000e+002 -3.9192000e+002  0.0000000e+000  1.7058070e+002  4.3715920e+002  6.6272540e+002  1.0113279e+003  1.4419546e+003  1.6470150e+003  1.7905570e+003  2.1107987e+003  2.4057380e+003  3.1155941e+003	
      | ]
  Gain : Gain  Gain=1.2  OutDataTypeStr=Inherit: Same as input  ParamDataTypeStr=Inherit: Same as input
  Lin/Spline switch : ManualSwitch
  Logical Operator : Logic  Operator=NOT  AllPortsSameDT=off  OutDataTypeStr=boolean
  Memory : Memory
  Minus1 : UnaryMinus
  Minus2 : UnaryMinus
  Product : Product  RndMeth=Zero  OutDataTypeStr=Inherit: Same as first input
  Product1 : Product  RndMeth=Zero  OutDataTypeStr=Inherit: Same as first input
  Vx Lookup : Lookup  InputValues=|  Table=|
      InputValues=|
      | [ -5e-2 -1e-2 -5e-3 0 5e-3 1e-2 5e-2
      | ]
      Table=|
      | [ 1 1 1 0.2 1 1 1
      | ]
  tag scope: FRDamperForce=global, InternalFRDamperActive=global
  wires:
  Data Type Conversion/1 -> [InternalFRDamperActive]
  Memory/1 -> Product/1
  Product/1 -> [FRDamperForce]
  Lin/Spline switch/1 -> Memory/1
  [FRDamperVelocity] -> Minus2/1, "C "/1
  Minus2/1 -> DmpF Lookup/1
  DmpF Lookup/1 -> Minus1/1
  "C "/1 -> Lin/Spline switch/2
  Minus1/1 -> Product1/2
  Product1/1 -> Lin/Spline switch/1
  Vx Lookup/1 -> Gain/1
  Gain/1 -> Product1/1
  [VerticalVelocity] -> Vx Lookup/1
  Constant/1 -> Product/2, Logical Operator/1
  Logical Operator/1 -> Data Type Conversion/1

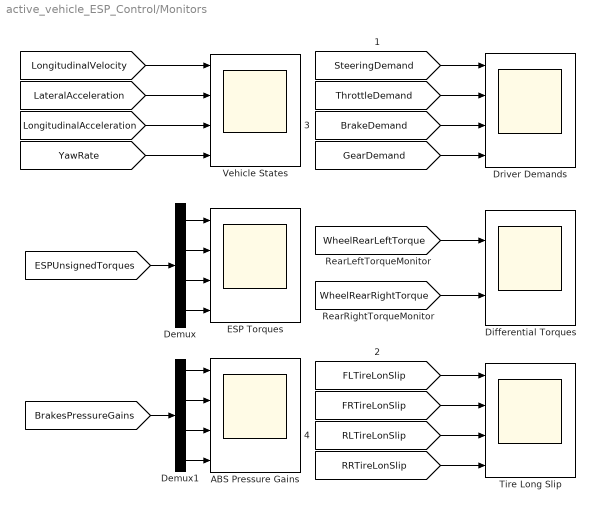
== system active_vehicle_ESP_Control/Monitors ==
  ABS Pressure Gains : Scope  NumInputPorts=4
  Demux : Demux
  Demux1 : Demux
  Differential Torques : Scope  NumInputPorts=2
  Driver Demands : Scope  NumInputPorts=4
  ESP Torques : Scope  NumInputPorts=4
  Tire Long Slip : Scope  NumInputPorts=4
  Vehicle States : Scope  NumInputPorts=4
  wires:
  [LongitudinalVelocity] -> Vehicle States/1
  [LateralAcceleration] -> Vehicle States/2
  [LongitudinalAcceleration] -> Vehicle States/3
  [YawRate] -> Vehicle States/4
  [SteeringDemand] -> Driver Demands/1
  [ThrottleDemand] -> Driver Demands/2
  [BrakeDemand] -> Driver Demands/3
  [GearDemand] -> Driver Demands/4
  [ESPUnsignedTorques] -> Demux/1
  Demux/1 -> ESP Torques/1
  Demux/2 -> ESP Torques/2
  Demux/3 -> ESP Torques/3
  Demux/4 -> ESP Torques/4
  Demux1/1 -> ABS Pressure Gains/1
  Demux1/2 -> ABS Pressure Gains/2
  Demux1/3 -> ABS Pressure Gains/3
  Demux1/4 -> ABS Pressure Gains/4
  [BrakesPressureGains] -> Demux1/1
  [FLTireLonSlip] -> Tire Long Slip/1
  [FRTireLonSlip] -> Tire Long Slip/2
  [RLTireLonSlip] -> Tire Long Slip/3
  [RRTireLonSlip] -> Tire Long Slip/4
  [WheelRearLeftTorque] -> Differential Torques/1
  [WheelRearRightTorque] -> Differential Torques/2

== system active_vehicle_ESP_Control/RL Damper ==
  "C " : Gain  Gain=4000  OutDataTypeStr=Inherit: Same as input  ParamDataTypeStr=Inherit: Same as input
  Constant : Constant  Value=RLDamperActive
  Data Type Conversion : DataTypeConversion
  DmpF Lookup : Lookup  InputValues=|  Table=|
      InputValues=|
      | [ -1.5800000e+000 -1.0200000e+000 -7.7000000e-001 -5.1000000e-001 -3.8000000e-001 -2.5000000e-001 -1.3000000e-001 -5.0000000e-002 -3.0000000e-002 -1.0000000e-002  0.0000000e+000  1.0000000e-002  3.0000000e-002  5.0000000e-002  1.3000000e-001  2.6000000e-001  3.8000000e-001  5.1000000e-001  7.8000000e-001  1.0400000e+000  1.6200000e+000	
      | ]
      Table=|
      | [ -3.2605700e+003 -2.6592520e+003 -2.3311553e+003 -1.9825529e+003 -1.7569865e+003 -1.5314201e+003 -1.2853477e+003 -8.9573310e+002 -7.0015000e+002 -3.9192000e+002  0.0000000e+000  1.7058070e+002  4.3715920e+002  6.6272540e+002  1.0113279e+003  1.4419546e+003  1.6470150e+003  1.7905570e+003  2.1107987e+003  2.4057380e+003  3.1155941e+003	
      | ]
  Gain : Gain  Gain=1.2  OutDataTypeStr=Inherit: Same as input  ParamDataTypeStr=Inherit: Same as input
  Lin/Spline switch : ManualSwitch
  Logical Operator : Logic  Operator=NOT  AllPortsSameDT=off  OutDataTypeStr=boolean
  Memory : Memory
  Minus1 : UnaryMinus
  Minus2 : UnaryMinus
  Product1 : Product  RndMeth=Zero  OutDataTypeStr=Inherit: Same as first input
  Product2 : Product  RndMeth=Zero  OutDataTypeStr=Inherit: Same as first input
  Scope : Scope
  Vx Lookup : Lookup  InputValues=|  Table=|
      InputValues=|
      | [ -5e-2 -1e-2 -5e-3 0 5e-3 1e-2 5e-2
      | ]
      Table=|
      | [ 1 1 1 0.2 1 1 1
      | ]
  tag scope: InternalRLDamperActive=global, RLDamperForce=global
  wires:
  Memory/1 -> Product2/1
  Product2/1 -> [RLDamperForce], Scope/1
  [RLDamperVelocity] -> Minus2/1, "C "/1
  Minus2/1 -> DmpF Lookup/1
  DmpF Lookup/1 -> Minus1/1
  "C "/1 -> Lin/Spline switch/2
  Lin/Spline switch/1 -> Memory/1
  Minus1/1 -> Product1/2
  Product1/1 -> Lin/Spline switch/1
  Vx Lookup/1 -> Gain/1
  Gain/1 -> Product1/1
  [VerticalVelocity] -> Vx Lookup/1
  Data Type Conversion/1 -> [InternalRLDamperActive]
  Constant/1 -> Product2/2, Logical Operator/1
  Logical Operator/1 -> Data Type Conversion/1

== system active_vehicle_ESP_Control/RR Damper ==
  "C " : Gain  Gain=4000  OutDataTypeStr=Inherit: Same as input  ParamDataTypeStr=Inherit: Same as input
  Constant : Constant  Value=RRDamperActive
  Data Type Conversion : DataTypeConversion
  DmpF Lookup : Lookup  InputValues=|  Table=|
      InputValues=|
      | [ -1.5800000e+000 -1.0200000e+000 -7.7000000e-001 -5.1000000e-001 -3.8000000e-001 -2.5000000e-001 -1.3000000e-001 -5.0000000e-002 -3.0000000e-002 -1.0000000e-002  0.0000000e+000  1.0000000e-002  3.0000000e-002  5.0000000e-002  1.3000000e-001  2.6000000e-001  3.8000000e-001  5.1000000e-001  7.8000000e-001  1.0400000e+000  1.6200000e+000	
      | ]
      Table=|
      | [ -3.2605700e+003 -2.6592520e+003 -2.3311553e+003 -1.9825529e+003 -1.7569865e+003 -1.5314201e+003 -1.2853477e+003 -8.9573310e+002 -7.0015000e+002 -3.9192000e+002  0.0000000e+000  1.7058070e+002  4.3715920e+002  6.6272540e+002  1.0113279e+003  1.4419546e+003  1.6470150e+003  1.7905570e+003  2.1107987e+003  2.4057380e+003  3.1155941e+003	
      | ]
  Gain : Gain  Gain=1.2  OutDataTypeStr=Inherit: Same as input  ParamDataTypeStr=Inherit: Same as input
  Lin/Spline switch : ManualSwitch
  Logical Operator : Logic  Operator=NOT  AllPortsSameDT=off  OutDataTypeStr=boolean
  Memory1 : Memory
  Minus1 : UnaryMinus
  Minus2 : UnaryMinus
  Product : Product  RndMeth=Zero  OutDataTypeStr=Inherit: Same as first input
  Product1 : Product  RndMeth=Zero  OutDataTypeStr=Inherit: Same as first input
  Vx Lookup : Lookup  InputValues=|  Table=|
      InputValues=|
      | [ -5e-2 -1e-2 -5e-3 0 5e-3 1e-2 5e-2
      | ]
      Table=|
      | [ 1 1 1 0.2 1 1 1
      | ]
  tag scope: InternalRRDamperActive=global, RRDamperForce=global
  wires:
  Product/1 -> [RRDamperForce]
  Memory1/1 -> Product/1
  Lin/Spline switch/1 -> Memory1/1
  [VerticalVelocity] -> Vx Lookup/1
  Gain/1 -> Product1/1
  Vx Lookup/1 -> Gain/1
  Product1/1 -> Lin/Spline switch/1
  Minus1/1 -> Product1/2
  "C "/1 -> Lin/Spline switch/2
  DmpF Lookup/1 -> Minus1/1
  Minus2/1 -> DmpF Lookup/1
  [RRDamperVelocity] -> Minus2/1, "C "/1
  Data Type Conversion/1 -> [InternalRRDamperActive]
  Constant/1 -> Product/2, Logical Operator/1
  Logical Operator/1 -> Data Type Conversion/1

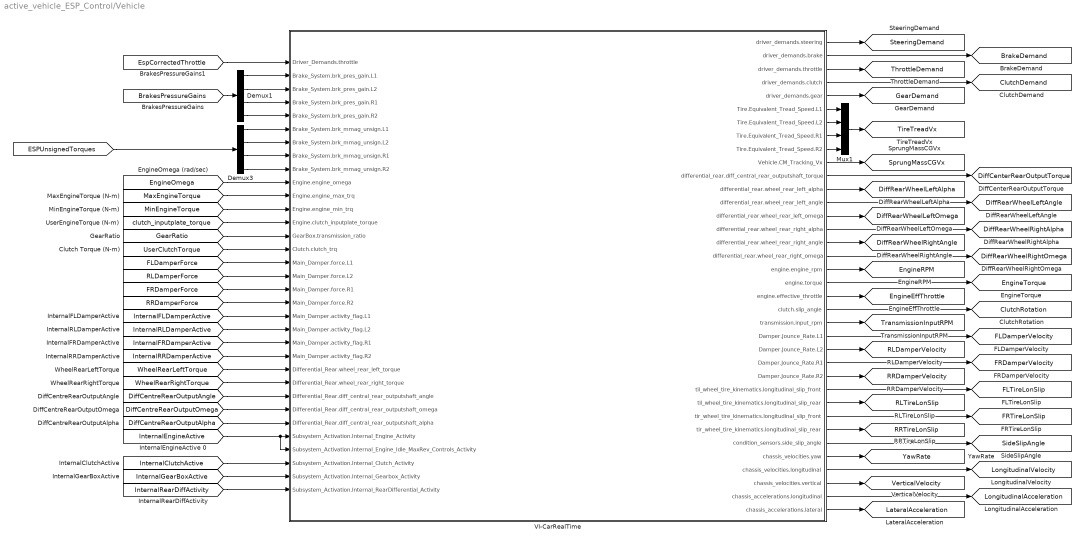
== system active_vehicle_ESP_Control/Vehicle ==
  Demux1 : Demux
  Demux3 : Demux
  Mux1 : Mux
  VI-CarRealTime : Subsystem  InitFcn=vicrt_simulationmanager(0);  TreatAsAtomicUnit=on
      mask help: Full VI-CarRealTime mex integrated with IO Bus
      settings: CopyFcn=set_param(gcb, 'LinkStatus', 'none');  ModelCloseFcn=vicrt_simulationmanager(2);  OpenFcn=vicrt_simulationmanager(1);
      mask Display: image(imread('vehicle.jpg'));color('red');port_label('input',1,'Driver_Demands.throttle');port_label('input',2,'Brake_System.brk_pres_gain.L1');port_label('input',3,'Brake_System.brk_pres_gain.L2');port_label('input',4,'Brake_System.brk_pres_gain.R1');port_label('input',5,'Brake_System.brk_pres_gain.R2');port_label('input',6,'Brake_System.brk_mmag_unsign.L1');port_label('input',7,'Brake_System.brk_mmag_unsign.L2');port_label('input',8,'Brake_System.brk_mmag_unsign.R1');port_label('input',9,'Brake_System.brk_mmag_unsign.R2');port_label('input',10,'Engine.engine_omega');port_label('input',11,'Engine.engine_max_trq');port_label('input',12,'Engine.engine_min_trq');port_label('input',13,'Engine.clutch_inputplate_torque');port_label('input',14,'GearBox.transmission_ratio');port_label('input',15,'Clutch.clutch_trq');port_label('input',16,'Main_Damper.force.L1');port_label('input',17,'Main_Damper.force.L2');port_label('input',18,'Main_Damper.force.R1');port_label('input',19,'Main_Damper.force.R2');port_label('input',20,'Main_Damper.activity_flag.L1');port_label('input',21,'Main_Damper.activity_flag.L2');port_label('input',22,'Main_Damper.activity_flag.R1');port_label('input',23,'Main_Damper.activity_flag.R2');port_label('input',24,'Differential_Rear.wheel_rear_left_torque');port_label('input',25,'Differential_Rear.wheel_rear_right_torque');port_label('input',26,'Differential_Rear.diff_central_rear_outputshaft_angle');port_label('input',27,'Differential_Rear.diff_central_rear_outputshaft_omega');port_label('input',28,'Differential_Rear.diff_central_rear_outputshaft_alpha');port_label('input',29,'Subsystem_Activation.Internal_Engine_Activity');port_label('input',30,'Subsystem_Activation.Internal_Engine_Idle_MaxRev_Controls_Activity');port_label('input',31,'Subsystem_Activation.Internal_Clutch_Activity');port_label('input',32,'Subsystem_Activation.Internal_Gearbox_Activity');port_label('input',33,'Subsystem_Activation.Internal_RearDifferential_Activity');port_label('output',1,'driver_demands.steering');port_label('output',2,'driver_demands.brake');port_label('output',3,'driver_demands.throttle');port_label('output',4,'driver_demands.clutch');port_label('output',5,'driver_demands.gear');port_label('output',6,'Tire.Equivalent_Tread_Speed.L1');port_label('output',7,'Tire.Equivalent_Tread_Speed.L2');port_label('output',8,'Tire.Equivalent_Tread_Speed.R1');port_label('output',9,'Tire.Equivalent_Tread_Speed.R2');port_label('output',10,'Vehicle.CM_Tracking_Vx');port_label('output',11,'differential_rear.diff_central_rear_outputshaft_torque');port_label('output',12,'differential_rear.wheel_rear_left_alpha');port_label('output',13,'differential_rear.wheel_rear_left_angle');port_label('output',14,'differential_rear.wheel_rear_left_omega');port_label('output',15,'differential_rear.wheel_rear_right_alpha');port_label('output',16,'differential_rear.wheel_rear_right_angle');port_label('output',17,'differential_rear.wheel_rear_right_omega');port_label('output',18,'engine.engine_rpm');port_label('output',19,'engine.torque');port_label('output',20,'engine.effective_throttle');port_label('output',21,'clutch.slip_angle');port_label('output',22,'transmission.input_rpm');port_label('output',23,'Damper.Jounce_Rate.L1');port_label('output',24,'Damper.Jounce_Rate.L2');port_label('output',25,'Damper.Jounce_Rate.R1');port_label('output',26,'Damper.Jounce_Rate.R2');port_label('output',27,'til_wheel_tire_kinematics.longitudinal_slip_front');port_label('output',28,'til_wheel_tire_kinematics.longitudinal_slip_rear');port_label('output',29,'tir_wheel_tire_kinematics.longitudinal_slip_front');port_label('output',30,'tir_wheel_tire_kinematics.longitudinal_slip_rear');port_label('output',31,'condition_sensors.side_slip_angle');port_label('output',32,'chassis_velocities.yaw');port_label('output',33,'chassis_velocities.longitudinal');port_label('output',34,'chassis_velocities.vertical');port_label('output',35,'chassis_accelerations.longitudinal');port_label('output',36,'chassis_accelerations.lateral');
  tag scope: BrakeDemand=global, ClutchDemand=global, ClutchRotation=global, DiffCenterRearOutputTorque=global, DiffRearWheelLeftAlpha=global, DiffRearWheelLeftAngle=global, DiffRearWheelLeftOmega=global, DiffRearWheelRightAlpha=global, DiffRearWheelRightAngle=global, DiffRearWheelRightOmega=global, EngineEffThrottle=global, EngineRPM=global, EngineTorque=global, FLDamperVelocity=global, FLTireLonSlip=global, FRDamperVelocity=global, FRTireLonSlip=global, GearDemand=global, LateralAcceleration=global, LongitudinalAcceleration=global, LongitudinalVelocity=global, RLDamperVelocity=global, RLTireLonSlip=global, RRDamperVelocity=global, RRTireLonSlip=global, SideSlipAngle=global, SprungMassCGVx=global, SteeringDemand=global, ThrottleDemand=global, TireTreadVx=global, TransmissionInputRPM=global, VerticalVelocity=global, YawRate=global
  wires:
  Mux1/1 -> [TireTreadVx]
  [BrakesPressureGains] -> Demux1/1
  [ESPUnsignedTorques] -> Demux3/1
  [EspCorrectedThrottle] -> VI-CarRealTime/1(Driver_Demands.throttle)
  Demux1/1 -> VI-CarRealTime/2(Brake_System.brk_pres_gain.L1)
  Demux1/2 -> VI-CarRealTime/3(Brake_System.brk_pres_gain.L2)
  Demux1/3 -> VI-CarRealTime/4(Brake_System.brk_pres_gain.R1)
  Demux1/4 -> VI-CarRealTime/5(Brake_System.brk_pres_gain.R2)
  Demux3/1 -> VI-CarRealTime/6(Brake_System.brk_mmag_unsign.L1)
  Demux3/2 -> VI-CarRealTime/7(Brake_System.brk_mmag_unsign.L2)
  Demux3/3 -> VI-CarRealTime/8(Brake_System.brk_mmag_unsign.R1)
  Demux3/4 -> VI-CarRealTime/9(Brake_System.brk_mmag_unsign.R2)
  [EngineOmega] -> VI-CarRealTime/10(Engine.engine_omega)
  [MaxEngineTorque] -> VI-CarRealTime/11(Engine.engine_max_trq)
  [MinEngineTorque] -> VI-CarRealTime/12(Engine.engine_min_trq)
  [clutch_inputplate_torque] -> VI-CarRealTime/13(Engine.clutch_inputplate_torque)
  [GearRatio] -> VI-CarRealTime/14(GearBox.transmission_ratio)
  [UserClutchTorque] -> VI-CarRealTime/15(Clutch.clutch_trq)
  [FLDamperForce] -> VI-CarRealTime/16(Main_Damper.force.L1)
  [RLDamperForce] -> VI-CarRealTime/17(Main_Damper.force.L2)
  [FRDamperForce] -> VI-CarRealTime/18(Main_Damper.force.R1)
  [RRDamperForce] -> VI-CarRealTime/19(Main_Damper.force.R2)
  [InternalFLDamperActive] -> VI-CarRealTime/20(Main_Damper.activity_flag.L1)
  [InternalRLDamperActive] -> VI-CarRealTime/21(Main_Damper.activity_flag.L2)
  [InternalFRDamperActive] -> VI-CarRealTime/22(Main_Damper.activity_flag.R1)
  [InternalRRDamperActive] -> VI-CarRealTime/23(Main_Damper.activity_flag.R2)
  [WheelRearLeftTorque] -> VI-CarRealTime/24(Differential_Rear.wheel_rear_left_torque)
  [WheelRearRightTorque] -> VI-CarRealTime/25(Differential_Rear.wheel_rear_right_torque)
  [DiffCentreRearOutputAngle] -> VI-CarRealTime/26(Differential_Rear.diff_central_rear_outputshaft_angle)
  [DiffCentreRearOutputOmega] -> VI-CarRealTime/27(Differential_Rear.diff_central_rear_outputshaft_omega)
  [DiffCentreRearOutputAlpha] -> VI-CarRealTime/28(Differential_Rear.diff_central_rear_outputshaft_alpha)
  [InternalEngineActive] -> VI-CarRealTime/30(Subsystem_Activation.Internal_Engine_Idle_MaxRev_Controls_Activity), VI-CarRealTime/29(Subsystem_Activation.Internal_Engine_Activity)
  [InternalClutchActive] -> VI-CarRealTime/31(Subsystem_Activation.Internal_Clutch_Activity)
  [InternalGearBoxActive] -> VI-CarRealTime/32(Subsystem_Activation.Internal_Gearbox_Activity)
  [InternalRearDiffActivity] -> VI-CarRealTime/33(Subsystem_Activation.Internal_RearDifferential_Activity)
  VI-CarRealTime/1(driver_demands.steering) -> [SteeringDemand]
  VI-CarRealTime/2(driver_demands.brake) -> [BrakeDemand]
  VI-CarRealTime/3(driver_demands.throttle) -> [ThrottleDemand]
  VI-CarRealTime/4(driver_demands.clutch) -> [ClutchDemand]
  VI-CarRealTime/5(driver_demands.gear) -> [GearDemand]
  VI-CarRealTime/6(Tire.Equivalent_Tread_Speed.L1) -> Mux1/1
  VI-CarRealTime/7(Tire.Equivalent_Tread_Speed.L2) -> Mux1/2
  VI-CarRealTime/8(Tire.Equivalent_Tread_Speed.R1) -> Mux1/3
  VI-CarRealTime/9(Tire.Equivalent_Tread_Speed.R2) -> Mux1/4
  VI-CarRealTime/10(Vehicle.CM_Tracking_Vx) -> [SprungMassCGVx]
  VI-CarRealTime/11(differential_rear.diff_central_rear_outputshaft_torque) -> [DiffCenterRearOutputTorque]
  VI-CarRealTime/12(differential_rear.wheel_rear_left_alpha) -> [DiffRearWheelLeftAlpha]
  VI-CarRealTime/13(differential_rear.wheel_rear_left_angle) -> [DiffRearWheelLeftAngle]
  VI-CarRealTime/14(differential_rear.wheel_rear_left_omega) -> [DiffRearWheelLeftOmega]
  VI-CarRealTime/15(differential_rear.wheel_rear_right_alpha) -> [DiffRearWheelRightAlpha]
  VI-CarRealTime/16(differential_rear.wheel_rear_right_angle) -> [DiffRearWheelRightAngle]
  VI-CarRealTime/17(differential_rear.wheel_rear_right_omega) -> [DiffRearWheelRightOmega]
  VI-CarRealTime/18(engine.engine_rpm) -> [EngineRPM]
  VI-CarRealTime/19(engine.torque) -> [EngineTorque]
  VI-CarRealTime/20(engine.effective_throttle) -> [EngineEffThrottle]
  VI-CarRealTime/21(clutch.slip_angle) -> [ClutchRotation]
  VI-CarRealTime/22(transmission.input_rpm) -> [TransmissionInputRPM]
  VI-CarRealTime/23(Damper.Jounce_Rate.L1) -> [FLDamperVelocity]
  VI-CarRealTime/24(Damper.Jounce_Rate.L2) -> [RLDamperVelocity]
  VI-CarRealTime/25(Damper.Jounce_Rate.R1) -> [FRDamperVelocity]
  VI-CarRealTime/26(Damper.Jounce_Rate.R2) -> [RRDamperVelocity]
  VI-CarRealTime/27(til_wheel_tire_kinematics.longitudinal_slip_front) -> [FLTireLonSlip]
  VI-CarRealTime/28(til_wheel_tire_kinematics.longitudinal_slip_rear) -> [RLTireLonSlip]
  VI-CarRealTime/29(tir_wheel_tire_kinematics.longitudinal_slip_front) -> [FRTireLonSlip]
  VI-CarRealTime/30(tir_wheel_tire_kinematics.longitudinal_slip_rear) -> [RRTireLonSlip]
  VI-CarRealTime/31(condition_sensors.side_slip_angle) -> [SideSlipAngle]
  VI-CarRealTime/32(chassis_velocities.yaw) -> [YawRate]
  VI-CarRealTime/33(chassis_velocities.longitudinal) -> [LongitudinalVelocity]
  VI-CarRealTime/34(chassis_velocities.vertical) -> [VerticalVelocity]
  VI-CarRealTime/35(chassis_accelerations.longitudinal) -> [LongitudinalAcceleration]
  VI-CarRealTime/36(chassis_accelerations.lateral) -> [LateralAcceleration]

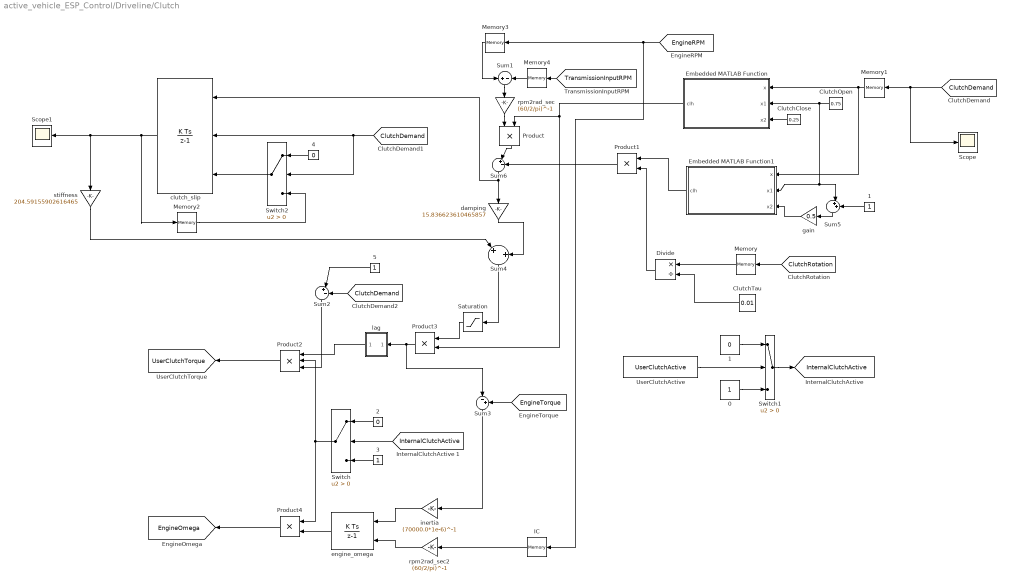
== system active_vehicle_ESP_Control/Driveline/Clutch ==
  {0..1,3,5} (4 alike) : Constant
  "1 " : Constant  Value=0
  2 : Constant  Value=0
  4 : Constant  Value=0
  ClutchClose : Constant  Value=0.25
  ClutchOpen : Constant  Value=0.75
  ClutchTau : Constant  Value=0.01
  Divide : Product  Inputs=*/  OutDataTypeStr=Inherit: Same as first input
  Embedded MATLAB Function : MATLAB Function  TreatAsAtomicUnit=on
  Embedded MATLAB Function1 : MATLAB Function  TreatAsAtomicUnit=on
  IC : Memory  InitialCondition=6027  InheritSampleTime=on
  Memory : Memory
  Memory1 : Memory
  Memory2 : Memory
  Memory3 : Memory  InitialCondition=6027  InheritSampleTime=on
  Memory4 : Memory  InitialCondition=6027  InheritSampleTime=on
  Product{,1,3..4} (4 alike) : Product  RndMeth=Zero  OutDataTypeStr=Inherit: Same as first input
  Product2 : Product  Inputs=3  RndMeth=Zero  OutDataTypeStr=Inherit: Same as first input
  Saturation : Saturate  UpperLimit=1000  LowerLimit=-1000
  Scope : Scope
  Scope1 : Scope
  Sum1 : Sum  Inputs=+-  OutDataTypeStr=Inherit: Same as first input
  Sum2 : Sum  Inputs=||+-  OutDataTypeStr=Inherit: Same as first input
  Sum3 : Sum  Inputs=|-+  OutDataTypeStr=Inherit: Same as first input
  Sum4 : Sum  Inputs=|+||+  OutDataTypeStr=Inherit: Same as first input
  Sum5 : Sum  Inputs=||++  OutDataTypeStr=Inherit: Same as first input
  Sum6 : Sum  Inputs=||+-  OutDataTypeStr=Inherit: Same as first input
  Switch : Switch  Criteria=u2 > Threshold
  Switch1 : Switch  Criteria=u2 > Threshold
  Switch2 : Switch  Criteria=u2 > Threshold
  UserClutchActive : Constant  Value=UserClutchActive
  clutch_slip : DiscreteIntegrator  ExternalReset=level  InitialConditionSource=external  SampleTime=-1  LowerSaturationLimit=-500  ICPrevOutput=DiscIntNeverNeededParam  ICPrevScaledInput=DiscIntNeverNeededParam
  damping : Gain  Gain=15.836623610465857  OutDataTypeStr=Inherit: Same as input  ParamDataTypeStr=Inherit: Same as input
  engine_omega : DiscreteIntegrator  InitialConditionSource=external  InitialCondition=600  SampleTime=-1  LowerSaturationLimit=1000/60*2*pi  ICPrevOutput=DiscIntNeverNeededParam  ICPrevScaledInput=DiscIntNeverNeededParam
  gain : Gain  Gain=0.5  OutDataTypeStr=Inherit: Same as input  ParamDataTypeStr=Inherit: Same as input
  inertia : Gain  Gain=(70000.0*1e-6)^-1  OutDataTypeStr=Inherit: Same as input  ParamDataTypeStr=Inherit: Same as input
  lag : Subsystem
  rpm2rad_sec : Gain  Gain=(60/2/pi)^-1  OutDataTypeStr=Inherit: Same as input  ParamDataTypeStr=Inherit: Same as input
  rpm2rad_sec2 : Gain  Gain=(60/2/pi)^-1  OutDataTypeStr=Inherit: Same as input  ParamDataTypeStr=Inherit: Same as input
  stiffness : Gain  Gain=204.59155902616465  OutDataTypeStr=Inherit: Same as input  ParamDataTypeStr=Inherit: Same as input
  tag scope: EngineOmega=global, InternalClutchActive=global, UserClutchTorque=global
  wires:
  [EngineRPM] -> Memory3/1, IC/1
  [TransmissionInputRPM] -> Memory4/1
  stiffness/1 -> Sum4/1
  damping/1 -> Sum4/2
  ClutchOpen/1 -> Embedded MATLAB Function/2(x1), Sum5/1, Embedded MATLAB Function1/2(x1)
  ClutchClose/1 -> Embedded MATLAB Function/3(x2)
  Embedded MATLAB Function/1(clh) -> Product/2, Product3/2
  Sum1/1 -> rpm2rad_sec/1
  1/1 -> Sum5/2
  Sum5/1 -> gain/1
  ClutchTau/1 -> Divide/2
  Divide/1 -> Product1/2
  Embedded MATLAB Function1/1(clh) -> Product1/1
  Product1/1 -> Sum6/2
  Sum6/1 -> damping/1, clutch_slip/1
  rpm2rad_sec/1 -> Product/1
  rpm2rad_sec2/1 -> engine_omega/2
  Product/1 -> Sum6/1
  Sum3/1 -> inertia/1
  inertia/1 -> engine_omega/1
  Memory/1 -> Divide/1
  Memory1/1 -> Embedded MATLAB Function1/1(x), Embedded MATLAB Function/1(x)
  gain/1 -> Embedded MATLAB Function1/3(x2)
  IC/1 -> rpm2rad_sec2/1
  Product3/1 -> Sum3/1, lag/1(In1)
  Memory3/1 -> Sum1/1
  Memory4/1 -> Sum1/2
  [ClutchRotation] -> Memory/1
  Saturation/1 -> Product3/1
  Sum4/1 -> Saturation/1
  Product2/1 -> [UserClutchTorque]
  Switch/1 -> Product2/2, Product4/1
  2/1 -> Switch/1
  [InternalClutchActive] -> Switch/2
  3/1 -> Switch/3
  engine_omega/1 -> Product4/2
  UserClutchActive/1 -> Switch1/2
  Switch1/1 -> [InternalClutchActive]
  "1 "/1 -> Switch1/1
  0/1 -> Switch1/3
  clutch_slip/1 -> Memory2/1, stiffness/1, Scope1/1
  [EngineTorque] -> Sum3/2
  Switch2/1 -> clutch_slip/3
  4/1 -> Switch2/1
  [ClutchDemand] -> Memory1/1, Scope/1
  lag/1(Out1) -> Product2/1
  Product4/1 -> [EngineOmega]
  5/1 -> Sum2/1
  Sum2/1 -> Product2/3
  [ClutchDemand] -> Switch2/2, clutch_slip/2
  [ClutchDemand] -> Sum2/2
  Memory2/1 -> Switch2/3

== system active_vehicle_ESP_Control/Driveline/Engine ==
  0 : Constant
  "1 " : Constant  Value=0
  Engine Maps : Subsystem
  Memory : Memory
  Product1 : Product  RndMeth=Zero  OutDataTypeStr=Inherit: Same as first input
  Product2 : Product  RndMeth=Zero  OutDataTypeStr=Inherit: Same as first input
  Sum : Sum  Inputs=+-  OutDataTypeStr=Inherit: Same as first input
  Switch1 : Switch  Criteria=u2 > Threshold
  ThrottleOff (from ESP) : Subsystem  mask{ThrottleOffScale=.1}
      mask prompts: ThrottleOffScale "Thottle Off Scale"
  UserEngineActive : Constant  Value=UserEngineActive
  tag scope: EspCorrectedThrottle=global, InternalEngineActive=global, MaxEngineTorque=global, MinEngineTorque=global, clutch_inputplate_torque=global
  wires:
  [EngineRPM] -> Engine Maps/1(RPM)
  [EngineEffThrottle] -> Memory/1
  Engine Maps/1(MaxEngineTorque) -> [MaxEngineTorque]
  Engine Maps/2(MinEngineTorque) -> [MinEngineTorque]
  Product1/1 -> Engine Maps/2(Throttle), Sum/1
  ThrottleOff (from ESP)/1(ThrottleGain) -> Product1/2
  Engine Maps/3(EngineTorque) -> [clutch_inputplate_torque]
  Sum/1 -> Product2/1
  [InternalEngineActive] -> Product2/2
  Product2/1 -> [EspCorrectedThrottle]
  Memory/1 -> Product1/1, Sum/2
  UserEngineActive/1 -> Switch1/2
  Switch1/1 -> [InternalEngineActive]
  "1 "/1 -> Switch1/1
  0/1 -> Switch1/3

== system active_vehicle_ESP_Control/Driveline/GearBox ==
  " " : Memory
  0 : Constant
  "1 " : Constant  Value=0
  Gear Ratio : Lookup  InputValues=[1 2 3 4 5 6]  Table=[2.88 1.77 1.27 1.0 0.88 0.71]
  Switch : Switch  Criteria=u2 > Threshold
  UserGearBoxActive : Constant  Value=UserGearBoxActive
  tag scope: GearRatio=global, InternalGearBoxActive=global
  wires:
  [GearDemand] -> " "/1
  Gear Ratio/1 -> [GearRatio]
  " "/1 -> Gear Ratio/1
  UserGearBoxActive/1 -> Switch/2
  Switch/1 -> [InternalGearBoxActive]
  "1 "/1 -> Switch/1
  0/1 -> Switch/3

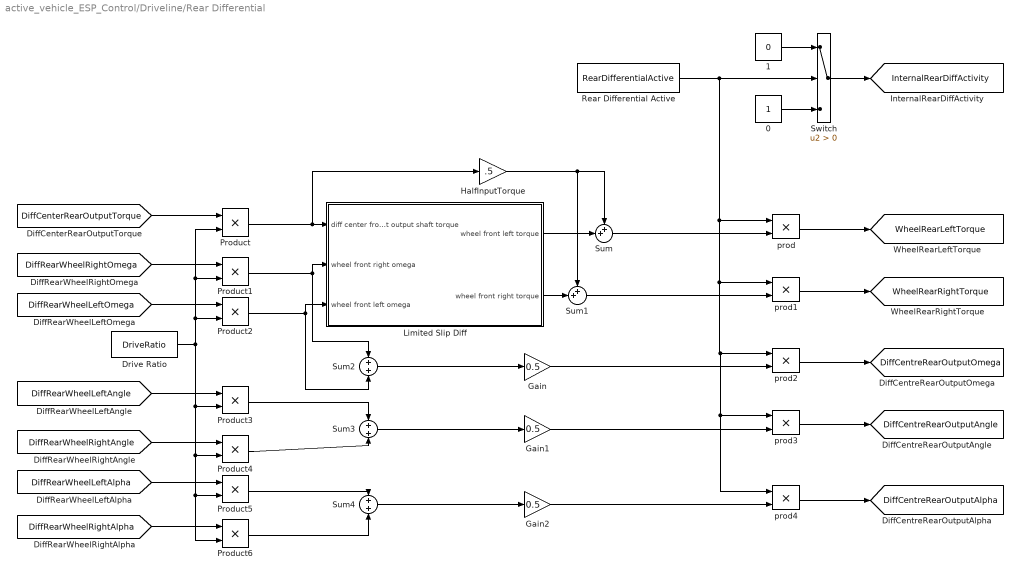
== system active_vehicle_ESP_Control/Driveline/Rear Differential ==
  0 : Constant
  "1 " : Constant  Value=0
  Drive Ratio : Constant  Value=DriveRatio
  Gain : Gain  Gain=0.5
  Gain1 : Gain  Gain=0.5
  Gain2 : Gain  Gain=0.5
  HalfInputTorque : Gain  Gain=.5
  Limited Slip Diff : Subsystem  mask{C0=0, C1=.2, C2=1.05, C3=1.1}
  Product{,1..6} (7 alike) : Product
  Rear Differential Active : Constant  Value=RearDifferentialActive
  Sum : Sum  Inputs=++|
  Sum1 : Sum  Inputs=++|
  Sum2 : Sum
  Sum3 : Sum
  Sum4 : Sum
  Switch : Switch  Criteria=u2 > Threshold
  prod{,1..4} (5 alike) : Product
  tag scope: DiffCentreRearOutputAlpha=global, DiffCentreRearOutputAngle=global, DiffCentreRearOutputOmega=global, InternalRearDiffActivity=global, WheelRearLeftTorque=global, WheelRearRightTorque=global
  wires:
  [DiffRearWheelRightAngle] -> Product4/1
  [DiffRearWheelLeftAlpha] -> Product5/1
  [DiffRearWheelLeftAngle] -> Product3/1
  Sum2/1 -> Gain/1
  [DiffRearWheelRightOmega] -> Product1/1
  [DiffRearWheelLeftOmega] -> Product2/1
  [DiffCenterRearOutputTorque] -> Product/1
  HalfInputTorque/1 -> Sum/1, Sum1/1
  Sum3/1 -> Gain1/1
  [DiffRearWheelRightAlpha] -> Product6/1
  Sum4/1 -> Gain2/1
  Limited Slip Diff/1(wheel front left torque) -> Sum/2
  Limited Slip Diff/2(wheel front right torque) -> Sum1/2
  Product/1 -> Limited Slip Diff/1(diff center front output shaft torque), HalfInputTorque/1
  Product1/1 -> Limited Slip Diff/2(wheel front right omega), Sum2/1
  Product2/1 -> Limited Slip Diff/3(wheel front left omega), Sum2/2
  Product3/1 -> Sum3/1
  Product4/1 -> Sum3/2
  Product5/1 -> Sum4/1
  Product6/1 -> Sum4/2
  Drive Ratio/1 -> Product6/2, Product5/2, Product4/2, Product3/2, Product2/2, Product1/2, Product/2
  Rear Differential Active/1 -> Switch/2, prod4/1, prod3/1, prod2/1, prod1/1, prod/1
  Sum/1 -> prod/2
  Sum1/1 -> prod1/2
  Gain/1 -> prod2/2
  Gain1/1 -> prod3/2
  Gain2/1 -> prod4/2
  Switch/1 -> [InternalRearDiffActivity]
  "1 "/1 -> Switch/1
  0/1 -> Switch/3
  prod/1 -> [WheelRearLeftTorque]
  prod1/1 -> [WheelRearRightTorque]
  prod2/1 -> [DiffCentreRearOutputOmega]
  prod3/1 -> [DiffCentreRearOutputAngle]
  prod4/1 -> [DiffCentreRearOutputAlpha]

== system active_vehicle_ESP_Control/ESP/ESP ==
  SIde_slip : Inport
  "yawr " : Inport  Port=2
  steer : Inport  Port=3
  Vx : Inport  Port=4
  Demux : Demux
  ESP Sensors : Scope  NumInputPorts=3
  Embedded MATLAB Function : MATLAB Function  TreatAsAtomicUnit=on
  Mux1 : Mux
  SteeringRatio : Constant  Value=SteeringRatio
  WheelBase : Constant  Value=WheelBase
  YawErrorToTorqueGain : Gain  Gain=[25 25 25 25]  OutDataTypeStr=Inherit: Same as input  ParamDataTypeStr=Inherit: Same as input
  LF : Outport
  LR : Outport  Port=2
  RF : Outport  Port=3
  RR : Outport  Port=4
  ThrottleOff : Outport  Port=5
  wires:
  Embedded MATLAB Function/7(yawrT) -> ESP Sensors/3
  Embedded MATLAB Function/5(overSteerRate) -> ESP Sensors/1
  YawErrorToTorqueGain/1 -> Demux/1
  Mux1/1 -> YawErrorToTorqueGain/1
  Embedded MATLAB Function/4(RR) -> Mux1/4
  Embedded MATLAB Function/3(RL) -> Mux1/3
  Embedded MATLAB Function/2(FR) -> Mux1/2
  Embedded MATLAB Function/1(FL) -> Mux1/1
  Demux/1 -> LF/1
  SIde_slip/1 -> Embedded MATLAB Function/1(SideSlip)
  Demux/2 -> RF/1
  Demux/3 -> LR/1
  steer/1 -> Embedded MATLAB Function/3(SWA)
  Demux/4 -> RR/1
  Vx/1 -> Embedded MATLAB Function/4(Vx)
  "yawr "/1 -> Embedded MATLAB Function/2(yawr)
  Embedded MATLAB Function/6(throttleOffTrigger) -> ThrottleOff/1, ESP Sensors/2
  WheelBase/1 -> Embedded MATLAB Function/5(WheelBase)
  SteeringRatio/1 -> Embedded MATLAB Function/6(steerRatio)

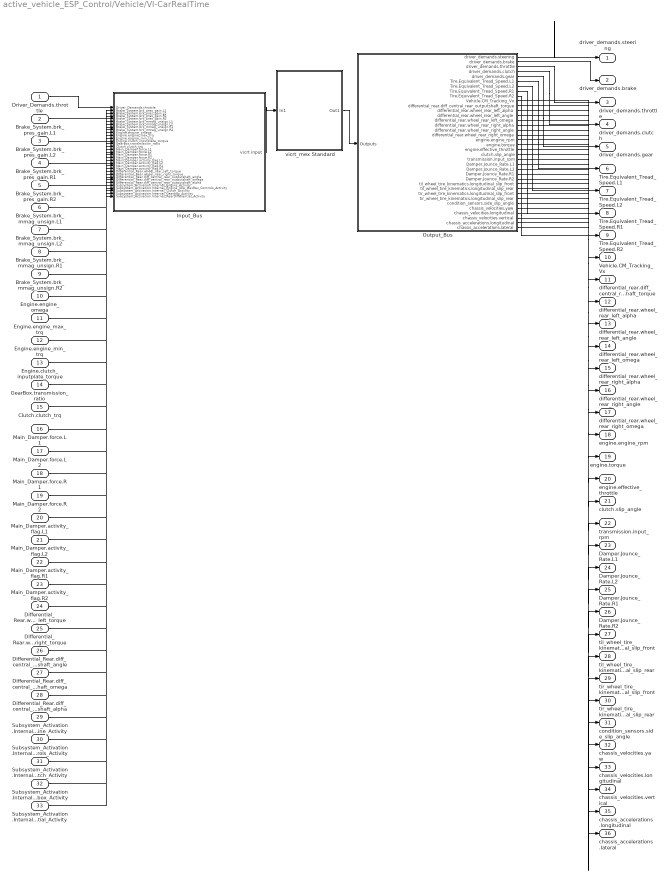
== system active_vehicle_ESP_Control/Vehicle/VI-CarRealTime ==
  Driver_Demands.throttle : Inport
  Brake_System.brk_pres_gain.L1 : Inport  Port=2
  Brake_System.brk_pres_gain.L2 : Inport  Port=3
  Brake_System.brk_pres_gain.R1 : Inport  Port=4
  Brake_System.brk_pres_gain.R2 : Inport  Port=5
  Brake_System.brk_mmag_unsign.L1 : Inport  Port=6
  Brake_System.brk_mmag_unsign.L2 : Inport  Port=7
  Brake_System.brk_mmag_unsign.R1 : Inport  Port=8
  Brake_System.brk_mmag_unsign.R2 : Inport  Port=9
  Engine.engine_omega : Inport  Port=10
  Engine.engine_max_trq : Inport  Port=11
  Engine.engine_min_trq : Inport  Port=12
  Engine.clutch_inputplate_torque : Inport  Port=13
  GearBox.transmission_ratio : Inport  Port=14
  Clutch.clutch_trq : Inport  Port=15
  Main_Damper.force.L1 : Inport  Port=16
  Main_Damper.force.L2 : Inport  Port=17
  Main_Damper.force.R1 : Inport  Port=18
  Main_Damper.force.R2 : Inport  Port=19
  Main_Damper.activity_flag.L1 : Inport  Port=20
  Main_Damper.activity_flag.L2 : Inport  Port=21
  Main_Damper.activity_flag.R1 : Inport  Port=22
  Main_Damper.activity_flag.R2 : Inport  Port=23
  Differential_Rear.wheel_rear_left_torque : Inport  Port=24
  Differential_Rear.wheel_rear_right_torque : Inport  Port=25
  Differential_Rear.diff_central_rear_outputshaft_angle : Inport  Port=26
  Differential_Rear.diff_central_rear_outputshaft_omega : Inport  Port=27
  Differential_Rear.diff_central_rear_outputshaft_alpha : Inport  Port=28
  Subsystem_Activation.Internal_Engine_Activity : Inport  Port=29
  Subsystem_Activation.Internal_Engine_Idle_MaxRev_Controls_Activity : Inport  Port=30
  Subsystem_Activation.Internal_Clutch_Activity : Inport  Port=31
  Subsystem_Activation.Internal_Gearbox_Activity : Inport  Port=32
  Subsystem_Activation.Internal_RearDifferential_Activity : Inport  Port=33
  Input_Bus : Subsystem  LoadFcn=vicrt_initcallback(gcb)
      settings: CopyFcn=vicrt_initcallback(gcb)
  Output_Bus : Subsystem  Description=Outputs
      settings: CopyFcn=set_param(gcb, 'LinkStatus', 'none')
  vicrt_mex Standard : Subsystem  mask{vicrt_inputfile=vicrt_inputfile, vicrt_outprefix='', intStep=0.001, AniFlag=on, inpPortDim=389, outPortDim=1374, NoDirectFeedthrough=on}
      mask prompts: vicrt_inputfile "VI-CarRealtime input file"; vicrt_outprefix "VI-CarRealTime output prefix"; intStep "Integration step"; AniFlag "live animation"; inpPortDim "input port dimension"; outPortDim "output port dimension"; NoDirectFeedthrough "Direct Feedthrough Off"
      mask init:
      | custDriv=[1,1,1];
      settings: CopyFcn=set_param(gcb, 'LinkStatus', 'none')
  driver_demands.steering : Outport
  driver_demands.brake : Outport  Port=2
  driver_demands.throttle : Outport  Port=3
  driver_demands.clutch : Outport  Port=4
  driver_demands.gear : Outport  Port=5
  Tire.Equivalent_Tread_Speed.L1 : Outport  Port=6
  Tire.Equivalent_Tread_Speed.L2 : Outport  Port=7
  Tire.Equivalent_Tread_Speed.R1 : Outport  Port=8
  Tire.Equivalent_Tread_Speed.R2 : Outport  Port=9
  Vehicle.CM_Tracking_Vx : Outport  Port=10
  differential_rear.diff_central_rear_outputshaft_torque : Outport  Port=11
  differential_rear.wheel_rear_left_alpha : Outport  Port=12
  differential_rear.wheel_rear_left_angle : Outport  Port=13
  differential_rear.wheel_rear_left_omega : Outport  Port=14
  differential_rear.wheel_rear_right_alpha : Outport  Port=15
  differential_rear.wheel_rear_right_angle : Outport  Port=16
  differential_rear.wheel_rear_right_omega : Outport  Port=17
  engine.engine_rpm : Outport  Port=18
  engine.torque : Outport  Port=19
  engine.effective_throttle : Outport  Port=20
  clutch.slip_angle : Outport  Port=21
  transmission.input_rpm : Outport  Port=22
  Damper.Jounce_Rate.L1 : Outport  Port=23
  Damper.Jounce_Rate.L2 : Outport  Port=24
  Damper.Jounce_Rate.R1 : Outport  Port=25
  Damper.Jounce_Rate.R2 : Outport  Port=26
  til_wheel_tire_kinematics.longitudinal_slip_front : Outport  Port=27
  til_wheel_tire_kinematics.longitudinal_slip_rear : Outport  Port=28
  tir_wheel_tire_kinematics.longitudinal_slip_front : Outport  Port=29
  tir_wheel_tire_kinematics.longitudinal_slip_rear : Outport  Port=30
  condition_sensors.side_slip_angle : Outport  Port=31
  chassis_velocities.yaw : Outport  Port=32
  chassis_velocities.longitudinal : Outport  Port=33
  chassis_velocities.vertical : Outport  Port=34
  chassis_accelerations.longitudinal : Outport  Port=35
  chassis_accelerations.lateral : Outport  Port=36
  wires:
  vicrt_mex Standard/1(Out1) -> Output_Bus/1(Outputs)
  Input_Bus/1(vicrt input) -> vicrt_mex Standard/1(In1)
  Driver_Demands.throttle/1 -> Input_Bus/1(Driver_Demands.throttle)
  Brake_System.brk_pres_gain.L1/1 -> Input_Bus/2(Brake_System.brk_pres_gain.L1)
  Brake_System.brk_pres_gain.L2/1 -> Input_Bus/3(Brake_System.brk_pres_gain.L2)
  Brake_System.brk_pres_gain.R1/1 -> Input_Bus/4(Brake_System.brk_pres_gain.R1)
  Brake_System.brk_pres_gain.R2/1 -> Input_Bus/5(Brake_System.brk_pres_gain.R2)
  Brake_System.brk_mmag_unsign.L1/1 -> Input_Bus/6(Brake_System.brk_mmag_unsign.L1)
  Brake_System.brk_mmag_unsign.L2/1 -> Input_Bus/7(Brake_System.brk_mmag_unsign.L2)
  Brake_System.brk_mmag_unsign.R1/1 -> Input_Bus/8(Brake_System.brk_mmag_unsign.R1)
  Brake_System.brk_mmag_unsign.R2/1 -> Input_Bus/9(Brake_System.brk_mmag_unsign.R2)
  Engine.engine_omega/1 -> Input_Bus/10(Engine.engine_omega)
  Engine.engine_max_trq/1 -> Input_Bus/11(Engine.engine_max_trq)
  Engine.engine_min_trq/1 -> Input_Bus/12(Engine.engine_min_trq)
  Engine.clutch_inputplate_torque/1 -> Input_Bus/13(Engine.clutch_inputplate_torque)
  GearBox.transmission_ratio/1 -> Input_Bus/14(GearBox.transmission_ratio)
  Clutch.clutch_trq/1 -> Input_Bus/15(Clutch.clutch_trq)
  Main_Damper.force.L1/1 -> Input_Bus/16(Main_Damper.force.L1)
  Main_Damper.force.L2/1 -> Input_Bus/17(Main_Damper.force.L2)
  Main_Damper.force.R1/1 -> Input_Bus/18(Main_Damper.force.R1)
  Main_Damper.force.R2/1 -> Input_Bus/19(Main_Damper.force.R2)
  Main_Damper.activity_flag.L1/1 -> Input_Bus/20(Main_Damper.activity_flag.L1)
  Main_Damper.activity_flag.L2/1 -> Input_Bus/21(Main_Damper.activity_flag.L2)
  Main_Damper.activity_flag.R1/1 -> Input_Bus/22(Main_Damper.activity_flag.R1)
  Main_Damper.activity_flag.R2/1 -> Input_Bus/23(Main_Damper.activity_flag.R2)
  Differential_Rear.wheel_rear_left_torque/1 -> Input_Bus/24(Differential_Rear.wheel_rear_left_torque)
  Differential_Rear.wheel_rear_right_torque/1 -> Input_Bus/25(Differential_Rear.wheel_rear_right_torque)
  Differential_Rear.diff_central_rear_outputshaft_angle/1 -> Input_Bus/26(Differential_Rear.diff_central_rear_outputshaft_angle)
  Differential_Rear.diff_central_rear_outputshaft_omega/1 -> Input_Bus/27(Differential_Rear.diff_central_rear_outputshaft_omega)
  Differential_Rear.diff_central_rear_outputshaft_alpha/1 -> Input_Bus/28(Differential_Rear.diff_central_rear_outputshaft_alpha)
  Subsystem_Activation.Internal_Engine_Activity/1 -> Input_Bus/29(Subsystem_Activation.Internal_Engine_Activity)
  Subsystem_Activation.Internal_Engine_Idle_MaxRev_Controls_Activity/1 -> Input_Bus/30(Subsystem_Activation.Internal_Engine_Idle_MaxRev_Controls_Activity)
  Subsystem_Activation.Internal_Clutch_Activity/1 -> Input_Bus/31(Subsystem_Activation.Internal_Clutch_Activity)
  Subsystem_Activation.Internal_Gearbox_Activity/1 -> Input_Bus/32(Subsystem_Activation.Internal_Gearbox_Activity)
  Subsystem_Activation.Internal_RearDifferential_Activity/1 -> Input_Bus/33(Subsystem_Activation.Internal_RearDifferential_Activity)
  Output_Bus/1(driver_demands.steering) -> driver_demands.steering/1
  Output_Bus/2(driver_demands.brake) -> driver_demands.brake/1
  Output_Bus/3(driver_demands.throttle) -> driver_demands.throttle/1
  Output_Bus/4(driver_demands.clutch) -> driver_demands.clutch/1
  Output_Bus/5(driver_demands.gear) -> driver_demands.gear/1
  Output_Bus/6(Tire.Equivalent_Tread_Speed.L1) -> Tire.Equivalent_Tread_Speed.L1/1
  Output_Bus/7(Tire.Equivalent_Tread_Speed.L2) -> Tire.Equivalent_Tread_Speed.L2/1
  Output_Bus/8(Tire.Equivalent_Tread_Speed.R1) -> Tire.Equivalent_Tread_Speed.R1/1
  Output_Bus/9(Tire.Equivalent_Tread_Speed.R2) -> Tire.Equivalent_Tread_Speed.R2/1
  Output_Bus/10(Vehicle.CM_Tracking_Vx) -> Vehicle.CM_Tracking_Vx/1
  Output_Bus/11(differential_rear.diff_central_rear_outputshaft_torque) -> differential_rear.diff_central_rear_outputshaft_torque/1
  Output_Bus/12(differential_rear.wheel_rear_left_alpha) -> differential_rear.wheel_rear_left_alpha/1
  Output_Bus/13(differential_rear.wheel_rear_left_angle) -> differential_rear.wheel_rear_left_angle/1
  Output_Bus/14(differential_rear.wheel_rear_left_omega) -> differential_rear.wheel_rear_left_omega/1
  Output_Bus/15(differential_rear.wheel_rear_right_alpha) -> differential_rear.wheel_rear_right_alpha/1
  Output_Bus/16(differential_rear.wheel_rear_right_angle) -> differential_rear.wheel_rear_right_angle/1
  Output_Bus/17(differential_rear.wheel_rear_right_omega) -> differential_rear.wheel_rear_right_omega/1
  Output_Bus/18(engine.engine_rpm) -> engine.engine_rpm/1
  Output_Bus/19(engine.torque) -> engine.torque/1
  Output_Bus/20(engine.effective_throttle) -> engine.effective_throttle/1
  Output_Bus/21(clutch.slip_angle) -> clutch.slip_angle/1
  Output_Bus/22(transmission.input_rpm) -> transmission.input_rpm/1
  Output_Bus/23(Damper.Jounce_Rate.L1) -> Damper.Jounce_Rate.L1/1
  Output_Bus/24(Damper.Jounce_Rate.L2) -> Damper.Jounce_Rate.L2/1
  Output_Bus/25(Damper.Jounce_Rate.R1) -> Damper.Jounce_Rate.R1/1
  Output_Bus/26(Damper.Jounce_Rate.R2) -> Damper.Jounce_Rate.R2/1
  Output_Bus/27(til_wheel_tire_kinematics.longitudinal_slip_front) -> til_wheel_tire_kinematics.longitudinal_slip_front/1
  Output_Bus/28(til_wheel_tire_kinematics.longitudinal_slip_rear) -> til_wheel_tire_kinematics.longitudinal_slip_rear/1
  Output_Bus/29(tir_wheel_tire_kinematics.longitudinal_slip_front) -> tir_wheel_tire_kinematics.longitudinal_slip_front/1
  Output_Bus/30(tir_wheel_tire_kinematics.longitudinal_slip_rear) -> tir_wheel_tire_kinematics.longitudinal_slip_rear/1
  Output_Bus/31(condition_sensors.side_slip_angle) -> condition_sensors.side_slip_angle/1
  Output_Bus/32(chassis_velocities.yaw) -> chassis_velocities.yaw/1
  Output_Bus/33(chassis_velocities.longitudinal) -> chassis_velocities.longitudinal/1
  Output_Bus/34(chassis_velocities.vertical) -> chassis_velocities.vertical/1
  Output_Bus/35(chassis_accelerations.longitudinal) -> chassis_accelerations.longitudinal/1
  Output_Bus/36(chassis_accelerations.lateral) -> chassis_accelerations.lateral/1

== system active_vehicle_ESP_Control/Driveline/Clutch/lag ==
  In1 : Inport
  Memory5 : Memory  InheritSampleTime=on
  Sum : Sum  Inputs=|++  OutDataTypeStr=Inherit: Same as first input
  "gain_1 " : Gain  Gain=1-exp(-2*pi*0.001)  OutDataTypeStr=Inherit: Same as input  ParamDataTypeStr=Inherit: Same as input
  gain_1 1 : Gain  Gain=exp(-2*pi*0.001)  OutDataTypeStr=Inherit: Same as input  ParamDataTypeStr=Inherit: Same as input
  Out1 : Outport
  wires:
  In1/1 -> "gain_1 "/1
  "gain_1 "/1 -> Sum/1
  Sum/1 -> Memory5/1, Out1/1
  Memory5/1 -> gain_1 1/1
  gain_1 1/1 -> Sum/2
